simulink model "ForwardKinematic_YuMi"  (R2024a)
(part 12 of 23)

(9007199067919185*sin(q2L)*((5557241208790345*cos(q1L))/9007199254740992 - (6384186990310915*sin(q1L))/9007199254740992))/9007199254740992 - 347859890694807798813742879236295256254610072729/24519928653854221733733552434404946937899825954937634816)))/36893488147419103232000 + (81222263116692158804177042061221826384594597321566869716687*((9007199067919185*cos(q4L))/9007199254740992 - (234819211581865*sin(q4L))/1152921504606846976)*((432094733372955093709245836907320566011451687275*cos(q1L))/2993155353253689176481146537402947624255349848014848 - (499823478647255911063139966257565597426350154025*cos(q2L))/1461501637330902918203684832716283019655932542976 + (376125364442766701270516501597006072214248637825*sin(q1L))/2993155353253689176481146537402947624255349848014848 - (67682029681889335677290557259385*cos(q2L)*((6384186990310915*cos(q1L))/9007199254740992 + (5557241208790345*sin(q1L))/9007199254740992))/332306998946228968225951765070086144 + (9007199067919185*sin(q2L)*((5557241208790345*cos(q1L))/9007199254740992 - (6384186990310915*sin(q1L))/9007199254740992))/9007199254740992 - 347859890694807798813742879236295256254610072729/24519928653854221733733552434404946937899825954937634816))/306499108173177771671669405430061836723747824436720435200000 + (81*((234819211581865*cos(q4L))/1152921504606846976 + (9007199067919185*sin(q4L))/9007199254740992)*((432094733372955093709245836907320566011451687275*cos(q1L))/2993155353253689176481146537402947624255349848014848 - (499823478647255911063139966257565597426350154025*cos(q2L))/1461501637330902918203684832716283019655932542976 + (376125364442766701270516501597006072214248637825*sin(q1L))/2993155353253689176481146537402947624255349848014848 - (67682029681889335677290557259385*cos(q2L)*((6384186990310915*cos(q1L))/9007199254740992 + (5557241208790345*sin(q1L))/9007199254740992))/332306998946228968225951765070086144 + (9007199067919185*sin(q2L)*((5557241208790345*cos(q1L))/9007199254740992 - (6384186990310915*sin(q1L))/9007199254740992))/9007199254740992 - 347859890694807798813742879236295256254610072729/24519928653854221733733552434404946937899825954937634816))/2000,(48638874966763599*cos(q5L)*((783310804561232573774573497517025067305577458842146606386579375*cos(q2L))/55213970774324510299478046898216203619608871777363092441300193790394368 - (677168015718420743488926864722853474412798830140650728756148125*cos(q1L))/113078212145816597093331040047546785012958969400039613319782796882727665664 - (589454226189876320500100500762517606499114263738369612804244375*sin(q1L))/113078212145816597093331040047546785012958969400039613319782796882727665664 + (106069577339469832923929692356850887620017617375*cos(q2L)*((6384186990310915*cos(q1L))/9007199254740992 + (5557241208790345*sin(q1L))/9007199254740992))/12554203470773361527671578846415332832204710888928069025792 - (14115856197532180673579726082375*sin(q2L)*((5557241208790345*cos(q1L))/9007199254740992 - (6384186990310915*sin(q1L))/9007199254740992))/340282366920938463463374607431768211456 + (67682029681889335677290557259385*cos(q3L)*((55491554575214198102159220722265*cos(q2L))/162259276829213363391578010288128 + (7514214926474921*cos(q2L)*((6384186990310915*cos(q1L))/9007199254740992 + (5557241208790345*sin(q1L))/9007199254740992))/36893488147419103232 - sin(q2L)*((5557241208790345*cos(q1L))/9007199254740992 - (6384186990310915*sin(q1L))/9007199254740992)))/332306998946228968225951765070086144 + (234819211581865*cos(q3L)*((55491554575214198102159220722265*sin(q2L))/162259276829213363391578010288128 + cos(q2L)*((5557241208790345*cos(q1L))/9007199254740992 - (6384186990310915*sin(q1L))/9007199254740992) + (7514214926474921*sin(q2L)*((6384186990310915*cos(q1L))/9007199254740992 + (5557241208790345*sin(q1L))/9007199254740992))/36893488147419103232))/1152921504606846976 - (1764482024691522628700660907665*sin(q3L)*((55491554575214198102159220722265*cos(q2L))/162259276829213363391578010288128 + (7514214926474921*cos(q2L)*((6384186990310915*cos(q1L))/9007199254740992 + (5557241208790345*sin(q1L))/9007199254740992))/36893488147419103232 - sin(q2L)*((5557241208790345*cos(q1L))/9007199254740992 - (6384186990310915*sin(q1L))/9007199254740992)))/42535295865117307932921825928971026432 + (81129635049124235038645691064225*cos(q3L)*((57503643108550260546605243404275*cos(q1L))/81129638414606681695789005144064 + (50055177836018480443110068268825*sin(q1L))/81129638414606681695789005144064 - 46293577452674263141823442369649/664613997892457936451903530140172288))/81129638414606681695789005144064 + (9007199067919185*sin(q3L)*((55491554575214198102159220722265*sin(q2L))/162259276829213363391578010288128 + cos(q2L)*((5557241208790345*cos(q1L))/9007199254740992 - (6384186990310915*sin(q1L))/9007199254740992) + (7514214926474921*sin(q2L)*((6384186990310915*cos(q1L))/9007199254740992 + (5557241208790345*sin(q1L))/9007199254740992))/36893488147419103232))/9007199254740992 - (2115063383689692319117831580025*sin(q3L)*((57503643108550260546605243404275*cos(q1L))/81129638414606681695789005144064 + (50055177836018480443110068268825*sin(q1L))/81129638414606681695789005144064 - 46293577452674263141823442369649/664613997892457936451903530140172288))/10384593717069655257060992658440192 + 545157285512458543963749743061519108960107968042455893206992575/926336713898529563388567880069503262826159877325124512315660672063305037119488))/1801439850948198400 + (170695144106365826517608855445768431563113584343*sin(q5L)*((783310804561232573774573497517025067305577458842146606386579375*cos(q2L))/55213970774324510299478046898216203619608871777363092441300193790394368 - (677168015718420743488926864722853474412798830140650728756148125*cos(q1L))/113078212145816597093331040047546785012958969400039613319782796882727665664 - (589454226189876320500100500762517606499114263738369612804244375*sin(q1L))/113078212145816597093331040047546785012958969400039613319782796882727665664 + (106069577339469832923929692356850887620017617375*cos(q2L)*((6384186990310915*cos(q1L))/9007199254740992 + (5557241208790345*sin(q1L))/9007199254740992))/12554203470773361527671578846415332832204710888928069025792 - (14115856197532180673579726082375*sin(q2L)*((5557241208790345*cos(q1L))/9007199254740992 - (6384186990310915*sin(q1L))/9007199254740992))/340282366920938463463374607431768211456 + (67682029681889335677290557259385*cos(q3L)*((55491554575214198102159220722265*cos(q2L))/162259276829213363391578010288128 + (7514214926474921*cos(q2L)*((6384186990310915*cos(q1L))/9007199254740992 + (5557241208790345*sin(q1L))/9007199254740992))/36893488147419103232 - sin(q2L)*((5557241208790345*cos(q1L))/9007199254740992 - (6384186990310915*sin(q1L))/9007199254740992)))/332306998946228968225951765070086144 + (234819211581865*cos(q3L)*((55491554575214198102159220722265*sin(q2L))/162259276829213363391578010288128 + cos(q2L)*((5557241208790345*cos(q1L))/9007199254740992 - (6384186990310915*sin(q1L))/9007199254740992) + (7514214926474921*sin(q2L)*((6384186990310915*cos(q1L))/9007199254740992 + (5557241208790345*sin(q1L))/9007199254740992))/36893488147419103232))/1152921504606846976 - (1764482024691522628700660907665*sin(q3L)*((55491554575214198102159220722265*cos(q2L))/162259276829213363391578010288128 + (7514214926474921*cos(q2L)*((6384186990310915*cos(q1L))/9007199254740992 + (5557241208790345*sin(q1L))/9007199254740992))/36893488147419103232 - sin(q2L)*((5557241208790345*cos(q1L))/9007199254740992 - (6384186990310915*sin(q1L))/9007199254740992)))/42535295865117307932921825928971026432 + (81129635049124235038645691064225*cos(q3L)*((57503643108550260546605243404275*cos(q1L))/81129638414606681695789005144064 + (50055177836018480443110068268825*sin(q1L))/81129638414606681695789005144064 - 46293577452674263141823442369649/664613997892457936451903530140172288))/81129638414606681695789005144064 + (9007199067919185*sin(q3L)*((55491554575214198102159220722265*sin(q2L))/162259276829213363391578010288128 + cos(q2L)*((5557241208790345*cos(q1L))/9007199254740992 - (6384186990310915*sin(q1L))/9007199254740992) + (7514214926474921*sin(q2L)*((6384186990310915*cos(q1L))/9007199254740992 + (5557241208790345*sin(q1L))/9007199254740992))/36893488147419103232))/9007199254740992 - (2115063383689692319117831580025*sin(q3L)*((57503643108550260546605243404275*cos(q1L))/81129638414606681695789005144064 + (50055177836018480443110068268825*sin(q1L))/81129638414606681695789005144064 - 46293577452674263141823442369649/664613997892457936451903530140172288))/10384593717069655257060992658440192 + 545157285512458543963749743061519108960107968042455893206992575/926336713898529563388567880069503262826159877325124512315660672063305037119488))/119726214130147567059245861496117904970213993920593920 - (27*cos(q6L)*((9007199067919185*cos(q5L)*((783310804561232573774573497517025067305577458842146606386579375*cos(q2L))/55213970774324510299478046898216203619608871777363092441300193790394368 - (677168015718420743488926864722853474412798830140650728756148125*cos(q1L))/113078212145816597093331040047546785012958969400039613319782796882727665664 - (589454226189876320500100500762517606499114263738369612804244375*sin(q1L))/113078212145816597093331040047546785012958969400039613319782796882727665664 + (106069577339469832923929692356850887620017617375*cos(q2L)*((6384186990310915*cos(q1L))/9007199254740992 + (5557241208790345*sin(q1L))/9007199254740992))/12554203470773361527671578846415332832204710888928069025792 - (14115856197532180673579726082375*sin(q2L)*((5557241208790345*cos(q1L))/9007199254740992 - (6384186990310915*sin(q1L))/9007199254740992))/340282366920938463463374607431768211456 + (67682029681889335677290557259385*cos(q3L)*((55491554575214198102159220722265*cos(q2L))/162259276829213363391578010288128 + (7514214926474921*cos(q2L)*((6384186990310915*cos(q1L))/9007199254740992 + (5557241208790345*sin(q1L))/9007199254740992))/36893488147419103232 - sin(q2L)*((5557241208790345*cos(q1L))/9007199254740992 - (6384186990310915*sin(q1L))/9007199254740992)))/332306998946228968225951765070086144 + (234819211581865*cos(q3L)*((55491554575214198102159220722265*sin(q2L))/162259276829213363391578010288128 + cos(q2L)*((5557241208790345*cos(q1L))/9007199254740992 - (6384186990310915*sin(q1L))/9007199254740992) + (7514214926474921*sin(q2L)*((6384186990310915*cos(q1L))/9007199254740992 + (5557241208790345*sin(q1L))/9007199254740992))/36893488147419103232))/1152921504606846976 - (1764482024691522628700660907665*sin(q3L)*((55491554575214198102159220722265*cos(q2L))/162259276829213363391578010288128 + (7514214926474921*cos(q2L)*((6384186990310915*cos(q1L))/9007199254740992 + (5557241208790345*sin(q1L))/9007199254740992))/36893488147419103232 - sin(q2L)*((5557241208790345*cos(q1L))/9007199254740992 - (6384186990310915*sin(q1L))/9007199254740992)))/42535295865117307932921825928971026432 + (81129635049124235038645691064225*cos(q3L)*((57503643108550260546605243404275*cos(q1L))/81129638414606681695789005144064 + (50055177836018480443110068268825*sin(q1L))/81129638414606681695789005144064 - 46293577452674263141823442369649/664613997892457936451903530140172288))/81129638414606681695789005144064 + (9007199067919185*sin(q3L)*((55491554575214198102159220722265*sin(q2L))/162259276829213363391578010288128 + cos(q2L)*((5557241208790345*cos(q1L))/9007199254740992 - (6384186990310915*sin(q1L))/9007199254740992) + (7514214926474921*sin(q2L)*((6384186990310915*cos(q1L))/9007199254740992 + (5557241208790345*sin(q1L))/9007199254740992))/36893488147419103232))/9007199254740992 - (2115063383689692319117831580025*sin(q3L)*((57503643108550260546605243404275*cos(q1L))/81129638414606681695789005144064 + (50055177836018480443110068268825*sin(q1L))/81129638414606681695789005144064 - 46293577452674263141823442369649/664613997892457936451903530140172288))/10384593717069655257060992658440192 + 545157285512458543963749743061519108960107968042455893206992575/926336713898529563388567880069503262826159877325124512315660672063305037119488))/9007199254740992 + (7514214926474921*cos(q5L)*((7514214926474921*cos(q4L)*((7514214926474921*cos(q3L)*((55491554575214198102159220722265*cos(q2L))/162259276829213363391578010288128 + (7514214926474921*cos(q2L)*((6384186990310915*cos(q1L))/9007199254740992 + (5557241208790345*sin(q1L))/9007199254740992))/36893488147419103232 - sin(q2L)*((5557241208790345*cos(q1L))/9007199254740992 - (6384186990310915*sin(q1L))/9007199254740992)))/36893488147419103232 + (9007199067919185*cos(q3L)*((57503643108550260546605243404275*cos(q1L))/81129638414606681695789005144064 + (50055177836018480443110068268825*sin(q1L))/81129638414606681695789005144064 - 46293577452674263141823442369649/664613997892457936451903530140172288))/9007199254740992 + sin(q3L)*((55491554575214198102159220722265*sin(q2L))/162259276829213363391578010288128 + cos(q2L)*((5557241208790345*cos(q1L))/9007199254740992 - (6384186990310915*sin(q1L))/9007199254740992) + (7514214926474921*sin(q2L)*((6384186990310915*cos(q1L))/9007199254740992 + (5557241208790345*sin(q1L))/9007199254740992))/36893488147419103232)))/36893488147419103232 + ((4503599440548691*cos(q4L))/4503599627370496 - (7514214926474921*sin(q4L))/36893488147419103232)*((7514214926474921*sin(q3L)*((55491554575214198102159220722265*cos(q2L))/162259276829213363391578010288128 + (7514214926474921*cos(q2L)*((6384186990310915*cos(q1L))/9007199254740992 + (5557241208790345*sin(q1L))/9007199254740992))/36893488147419103232 - sin(q2L)*((5557241208790345*cos(q1L))/9007199254740992 - (6384186990310915*sin(q1L))/9007199254740992)))/36893488147419103232 - cos(q3L)*((55491554575214198102159220722265*sin(q2L))/162259276829213363391578010288128 + cos(q2L)*((5557241208790345*cos(q1L))/9007199254740992 - (6384186990310915*sin(q1L))/9007199254740992) + (7514214926474921*sin(q2L)*((6384186990310915*cos(q1L))/9007199254740992 + (5557241208790345*sin(q1L))/9007199254740992))/36893488147419103232) + (9007199067919185*sin(q3L)*((57503643108550260546605243404275*cos(q1L))/81129638414606681695789005144064 + (50055177836018480443110068268825*sin(q1L))/81129638414606681695789005144064 - 46293577452674263141823442369649/664613997892457936451903530140172288))/9007199254740992) + ((234819211581865*cos(q4L))/1152921504606846976 + (9007199067919185*sin(q4L))/9007199254740992)*((432094733372955093709245836907320566011451687275*cos(q1L))/2993155353253689176481146537402947624255349848014848 - (499823478647255911063139966257565597426350154025*cos(q2L))/1461501637330902918203684832716283019655932542976 + (376125364442766701270516501597006072214248637825*sin(q1L))/2993155353253689176481146537402947624255349848014848 - (67682029681889335677290557259385*cos(q2L)*((6384186990310915*cos(q1L))/9007199254740992 + (5557241208790345*sin(q1L))/9007199254740992))/332306998946228968225951765070086144 + (9007199067919185*sin(q2L)*((5557241208790345*cos(q1L))/9007199254740992 - (6384186990310915*sin(q1L))/9007199254740992))/9007199254740992 - 347859890694807798813742879236295256254610072729/24519928653854221733733552434404946937899825954937634816)))/36893488147419103232 + sin(q5L)*((7514214926474921*sin(q4L)*((7514214926474921*cos(q3L)*((55491554575214198102159220722265*cos(q2L))/162259276829213363391578010288128 + (7514214926474921*cos(q2L)*((6384186990310915*cos(q1L))/9007199254740992 + (5557241208790345*sin(q1L))/9007199254740992))/36893488147419103232 - sin(q2L)*((5557241208790345*cos(q1L))/9007199254740992 - (6384186990310915*sin(q1L))/9007199254740992)))/36893488147419103232 + (9007199067919185*cos(q3L)*((57503643108550260546605243404275*cos(q1L))/81129638414606681695789005144064 + (50055177836018480443110068268825*sin(q1L))/81129638414606681695789005144064 - 46293577452674263141823442369649/664613997892457936451903530140172288))/9007199254740992 + sin(q3L)*((55491554575214198102159220722265*sin(q2L))/162259276829213363391578010288128 + cos(q2L)*((5557241208790345*cos(q1L))/9007199254740992 - (6384186990310915*sin(q1L))/9007199254740992) + (7514214926474921*sin(q2L)*((6384186990310915*cos(q1L))/9007199254740992 + (5557241208790345*sin(q1L))/9007199254740992))/36893488147419103232)))/36893488147419103232 + ((7514214926474921*cos(q4L))/36893488147419103232 + (4503599440548691*sin(q4L))/4503599627370496)*((7514214926474921*sin(q3L)*((55491554575214198102159220722265*cos(q2L))/162259276829213363391578010288128 + (7514214926474921*cos(q2L)*((6384186990310915*cos(q1L))/9007199254740992 + (5557241208790345*sin(q1L))/9007199254740992))/36893488147419103232 - sin(q2L)*((5557241208790345*cos(q1L))/9007199254740992 - (6384186990310915*sin(q1L))/9007199254740992)))/36893488147419103232 - cos(q3L)*((55491554575214198102159220722265*sin(q2L))/162259276829213363391578010288128 + cos(q2L)*((5557241208790345*cos(q1L))/9007199254740992 - (6384186990310915*sin(q1L))/9007199254740992) + (7514214926474921*sin(q2L)*((6384186990310915*cos(q1L))/9007199254740992 + (5557241208790345*sin(q1L))/9007199254740992))/36893488147419103232) + (9007199067919185*sin(q3L)*((57503643108550260546605243404275*cos(q1L))/81129638414606681695789005144064 + (50055177836018480443110068268825*sin(q1L))/81129638414606681695789005144064 - 46293577452674263141823442369649/664613997892457936451903530140172288))/9007199254740992) - ((9007199067919185*cos(q4L))/9007199254740992 - (234819211581865*sin(q4L))/1152921504606846976)*((432094733372955093709245836907320566011451687275*cos(q1L))/2993155353253689176481146537402947624255349848014848 - (499823478647255911063139966257565597426350154025*cos(q2L))/1461501637330902918203684832716283019655932542976 + (376125364442766701270516501597006072214248637825*sin(q1L))/2993155353253689176481146537402947624255349848014848 - (67682029681889335677290557259385*cos(q2L)*((6384186990310915*cos(q1L))/9007199254740992 + (5557241208790345*sin(q1L))/9007199254740992))/332306998946228968225951765070086144 + (9007199067919185*sin(q2L)*((5557241208790345*cos(q1L))/9007199254740992 - (6384186990310915*sin(q1L))/9007199254740992))/9007199254740992 - 347859890694807798813742879236295256254610072729/24519928653854221733733552434404946937899825954937634816))))/1000 + (324259171862923063*sin(q6L)*((9007199067919185*cos(q5L)*((783310804561232573774573497517025067305577458842146606386579375*cos(q2L))/55213970774324510299478046898216203619608871777363092441300193790394368 - (677168015718420743488926864722853474412798830140650728756148125*cos(q1L))/113078212145816597093331040047546785012958969400039613319782796882727665664 - (589454226189876320500100500762517606499114263738369612804244375*sin(q1L))/113078212145816597093331040047546785012958969400039613319782796882727665664 + (106069577339469832923929692356850887620017617375*cos(q2L)*((6384186990310915*cos(q1L))/9007199254740992 + (5557241208790345*sin(q1L))/9007199254740992))/12554203470773361527671578846415332832204710888928069025792 - (14115856197532180673579726082375*sin(q2L)*((5557241208790345*cos(q1L))/9007199254740992 - (6384186990310915*sin(q1L))/9007199254740992))/340282366920938463463374607431768211456 + (67682029681889335677290557259385*cos(q3L)*((55491554575214198102159220722265*cos(q2L))/162259276829213363391578010288128 + (7514214926474921*cos(q2L)*((6384186990310915*cos(q1L))/9007199254740992 + (5557241208790345*sin(q1L))/9007199254740992))/36893488147419103232 - sin(q2L)*((5557241208790345*cos(q1L))/9007199254740992 - (6384186990310915*sin(q1L))/9007199254740992)))/332306998946228968225951765070086144 + (234819211581865*cos(q3L)*((55491554575214198102159220722265*sin(q2L))/162259276829213363391578010288128 + cos(q2L)*((5557241208790345*cos(q1L))/9007199254740992 - (6384186990310915*sin(q1L))/9007199254740992) + (7514214926474921*sin(q2L)*((6384186990310915*cos(q1L))/9007199254740992 + (5557241208790345*sin(q1L))/9007199254740992))/36893488147419103232))/1152921504606846976 - (1764482024691522628700660907665*sin(q3L)*((55491554575214198102159220722265*cos(q2L))/162259276829213363391578010288128 + (7514214926474921*cos(q2L)*((6384186990310915*cos(q1L))/9007199254740992 + (5557241208790345*sin(q1L))/9007199254740992))/36893488147419103232 - sin(q2L)*((5557241208790345*cos(q1L))/9007199254740992 - (6384186990310915*sin(q1L))/9007199254740992)))/42535295865117307932921825928971026432 + (81129635049124235038645691064225*cos(q3L)*((57503643108550260546605243404275*cos(q1L))/81129638414606681695789005144064 + (50055177836018480443110068268825*sin(q1L))/81129638414606681695789005144064 - 46293577452674263141823442369649/664613997892457936451903530140172288))/81129638414606681695789005144064 + (9007199067919185*sin(q3L)*((55491554575214198102159220722265*sin(q2L))/162259276829213363391578010288128 + cos(q2L)*((5557241208790345*cos(q1L))/9007199254740992 - (6384186990310915*sin(q1L))/9007199254740992) + (7514214926474921*sin(q2L)*((6384186990310915*cos(q1L))/9007199254740992 + (5557241208790345*sin(q1L))/9007199254740992))/36893488147419103232))/9007199254740992 - (2115063383689692319117831580025*sin(q3L)*((57503643108550260546605243404275*cos(q1L))/81129638414606681695789005144064 + (50055177836018480443110068268825*sin(q1L))/81129638414606681695789005144064 - 46293577452674263141823442369649/664613997892457936451903530140172288))/10384593717069655257060992658440192 + 545157285512458543963749743061519108960107968042455893206992575/926336713898529563388567880069503262826159877325124512315660672063305037119488))/9007199254740992 + (7514214926474921*cos(q5L)*((7514214926474921*cos(q4L)*((7514214926474921*cos(q3L)*((55491554575214198102159220722265*cos(q2L))/162259276829213363391578010288128 + (7514214926474921*cos(q2L)*((6384186990310915*cos(q1L))/9007199254740992 + (5557241208790345*sin(q1L))/9007199254740992))/36893488147419103232 - sin(q2L)*((5557241208790345*cos(q1L))/9007199254740992 - (6384186990310915*sin(q1L))/9007199254740992)))/36893488147419103232 + (9007199067919185*cos(q3L)*((57503643108550260546605243404275*cos(q1L))/81129638414606681695789005144064 + (50055177836018480443110068268825*sin(q1L))/81129638414606681695789005144064 - 46293577452674263141823442369649/664613997892457936451903530140172288))/9007199254740992 + sin(q3L)*((55491554575214198102159220722265*sin(q2L))/162259276829213363391578010288128 + cos(q2L)*((5557241208790345*cos(q1L))/9007199254740992 - (6384186990310915*sin(q1L))/9007199254740992) + (7514214926474921*sin(q2L)*((6384186990310915*cos(q1L))/9007199254740992 + (5557241208790345*sin(q1L))/9007199254740992))/36893488147419103232)))/36893488147419103232 + ((4503599440548691*cos(q4L))/4503599627370496 - (7514214926474921*sin(q4L))/36893488147419103232)*((7514214926474921*sin(q3L)*((55491554575214198102159220722265*cos(q2L))/162259276829213363391578010288128 + (7514214926474921*cos(q2L)*((6384186990310915*cos(q1L))/9007199254740992 + (5557241208790345*sin(q1L))/9007199254740992))/36893488147419103232 - sin(q2L)*((5557241208790345*cos(q1L))/9007199254740992 - (6384186990310915*sin(q1L))/9007199254740992)))/36893488147419103232 - cos(q3L)*((55491554575214198102159220722265*sin(q2L))/162259276829213363391578010288128 + cos(q2L)*((5557241208790345*cos(q1L))/9007199254740992 - (6384186990310915*sin(q1L))/9007199254740992) + (7514214926474921*sin(q2L)*((6384186990310915*cos(q1L))/9007199254740992 + (5557241208790345*sin(q1L))/9007199254740992))/36893488147419103232) + (9007199067919185*sin(q3L)*((57503643108550260546605243404275*cos(q1L))/81129638414606681695789005144064 + (50055177836018480443110068268825*sin(q1L))/81129638414606681695789005144064 - 46293577452674263141823442369649/664613997892457936451903530140172288))/9007199254740992) + ((234819211581865*cos(q4L))/1152921504606846976 + (9007199067919185*sin(q4L))/9007199254740992)*((432094733372955093709245836907320566011451687275*cos(q1L))/2993155353253689176481146537402947624255349848014848 - (499823478647255911063139966257565597426350154025*cos(q2L))/1461501637330902918203684832716283019655932542976 + (376125364442766701270516501597006072214248637825*sin(q1L))/2993155353253689176481146537402947624255349848014848 - (67682029681889335677290557259385*cos(q2L)*((6384186990310915*cos(q1L))/9007199254740992 + (5557241208790345*sin(q1L))/9007199254740992))/332306998946228968225951765070086144 + (9007199067919185*sin(q2L)*((5557241208790345*cos(q1L))/9007199254740992 - (6384186990310915*sin(q1L))/9007199254740992))/9007199254740992 - 347859890694807798813742879236295256254610072729/24519928653854221733733552434404946937899825954937634816)))/36893488147419103232 + sin(q5L)*((7514214926474921*sin(q4L)*((7514214926474921*cos(q3L)*((55491554575214198102159220722265*cos(q2L))/162259276829213363391578010288128 + (7514214926474921*cos(q2L)*((6384186990310915*cos(q1L))/9007199254740992 + (5557241208790345*sin(q1L))/9007199254740992))/36893488147419103232 - sin(q2L)*((5557241208790345*cos(q1L))/9007199254740992 - (6384186990310915*sin(q1L))/9007199254740992)))/36893488147419103232 + (9007199067919185*cos(q3L)*((57503643108550260546605243404275*cos(q1L))/81129638414606681695789005144064 + (50055177836018480443110068268825*sin(q1L))/81129638414606681695789005144064 - 46293577452674263141823442369649/664613997892457936451903530140172288))/9007199254740992 + sin(q3L)*((55491554575214198102159220722265*sin(q2L))/162259276829213363391578010288128 + cos(q2L)*((5557241208790345*cos(q1L))/9007199254740992 - (6384186990310915*sin(q1L))/9007199254740992) + (7514214926474921*sin(q2L)*((6384186990310915*cos(q1L))/9007199254740992 + (5557241208790345*sin(q1L))/9007199254740992))/36893488147419103232)))/36893488147419103232 + ((7514214926474921*cos(q4L))/36893488147419103232 + (4503599440548691*sin(q4L))/4503599627370496)*((7514214926474921*sin(q3L)*((55491554575214198102159220722265*cos(q2L))/162259276829213363391578010288128 + (7514214926474921*cos(q2L)*((6384186990310915*cos(q1L))/9007199254740992 + (5557241208790345*sin(q1L))/9007199254740992))/36893488147419103232 - sin(q2L)*((5557241208790345*cos(q1L))/9007199254740992 - (6384186990310915*sin(q1L))/9007199254740992)))/36893488147419103232 - cos(q3L)*((55491554575214198102159220722265*sin(q2L))/162259276829213363391578010288128 + cos(q2L)*((5557241208790345*cos(q1L))/9007199254740992 - (6384186990310915*sin(q1L))/9007199254740992) + (7514214926474921*sin(q2L)*((6384186990310915*cos(q1L))/9007199254740992 + (5557241208790345*sin(q1L))/9007199254740992))/36893488147419103232) + (9007199067919185*sin(q3L)*((57503643108550260546605243404275*cos(q1L))/81129638414606681695789005144064 + (50055177836018480443110068268825*sin(q1L))/81129638414606681695789005144064 - 46293577452674263141823442369649/664613997892457936451903530140172288))/9007199254740992) - ((9007199067919185*cos(q4L))/9007199254740992 - (234819211581865*sin(q4L))/1152921504606846976)*((432094733372955093709245836907320566011451687275*cos(q1L))/2993155353253689176481146537402947624255349848014848 - (499823478647255911063139966257565597426350154025*cos(q2L))/1461501637330902918203684832716283019655932542976 + (376125364442766701270516501597006072214248637825*sin(q1L))/2993155353253689176481146537402947624255349848014848 - (67682029681889335677290557259385*cos(q2L)*((6384186990310915*cos(q1L))/9007199254740992 + (5557241208790345*sin(q1L))/9007199254740992))/332306998946228968225951765070086144 + (9007199067919185*sin(q2L)*((5557241208790345*cos(q1L))/9007199254740992 - (6384186990310915*sin(q1L))/9007199254740992))/9007199254740992 - 347859890694807798813742879236295256254610072729/24519928653854221733733552434404946937899825954937634816))))/9007199254740992000 - (2436553109258773196144549622003023*cos(q6L)*((9007199067919185*sin(q5L)*((783310804561232573774573497517025067305577458842146606386579375*cos(q2L))/55213970774324510299478046898216203619608871777363092441300193790394368 - (677168015718420743488926864722853474412798830140650728756148125*cos(q1L))/113078212145816597093331040047546785012958969400039613319782796882727665664 - (589454226189876320500100500762517606499114263738369612804244375*sin(q1L))/113078212145816597093331040047546785012958969400039613319782796882727665664 + (106069577339469832923929692356850887620017617375*cos(q2L)*((6384186990310915*cos(q1L))/9007199254740992 + (5557241208790345*sin(q1L))/9007199254740992))/12554203470773361527671578846415332832204710888928069025792 - (14115856197532180673579726082375*sin(q2L)*((5557241208790345*cos(q1L))/9007199254740992 - (6384186990310915*sin(q1L))/9007199254740992))/340282366920938463463374607431768211456 + (67682029681889335677290557259385*cos(q3L)*((55491554575214198102159220722265*cos(q2L))/162259276829213363391578010288128 + (7514214926474921*cos(q2L)*((6384186990310915*cos(q1L))/9007199254740992 + (5557241208790345*sin(q1L))/9007199254740992))/36893488147419103232 - sin(q2L)*((5557241208790345*cos(q1L))/9007199254740992 - (6384186990310915*sin(q1L))/9007199254740992)))/332306998946228968225951765070086144 + (234819211581865*cos(q3L)*((55491554575214198102159220722265*sin(q2L))/162259276829213363391578010288128 + cos(q2L)*((5557241208790345*cos(q1L))/9007199254740992 - (6384186990310915*sin(q1L))/9007199254740992) + (7514214926474921*sin(q2L)*((6384186990310915*cos(q1L))/9007199254740992 + (5557241208790345*sin(q1L))/9007199254740992))/36893488147419103232))/1152921504606846976 - (1764482024691522628700660907665*sin(q3L)*((55491554575214198102159220722265*cos(q2L))/162259276829213363391578010288128 + (7514214926474921*cos(q2L)*((6384186990310915*cos(q1L))/9007199254740992 + (5557241208790345*sin(q1L))/9007199254740992))/36893488147419103232 - sin(q2L)*((5557241208790345*cos(q1L))/9007199254740992 - (6384186990310915*sin(q1L))/9007199254740992)))/42535295865117307932921825928971026432 + (81129635049124235038645691064225*cos(q3L)*((57503643108550260546605243404275*cos(q1L))/81129638414606681695789005144064 + (50055177836018480443110068268825*sin(q1L))/81129638414606681695789005144064 - 46293577452674263141823442369649/664613997892457936451903530140172288))/81129638414606681695789005144064 + (9007199067919185*sin(q3L)*((55491554575214198102159220722265*sin(q2L))/162259276829213363391578010288128 + cos(q2L)*((5557241208790345*cos(q1L))/9007199254740992 - (6384186990310915*sin(q1L))/9007199254740992) + (7514214926474921*sin(q2L)*((6384186990310915*cos(q1L))/9007199254740992 + (5557241208790345*sin(q1L))/9007199254740992))/36893488147419103232))/9007199254740992 - (2115063383689692319117831580025*sin(q3L)*((57503643108550260546605243404275*cos(q1L))/81129638414606681695789005144064 + (50055177836018480443110068268825*sin(q1L))/81129638414606681695789005144064 - 46293577452674263141823442369649/664613997892457936451903530140172288))/10384593717069655257060992658440192 + 545157285512458543963749743061519108960107968042455893206992575/926336713898529563388567880069503262826159877325124512315660672063305037119488))/9007199254740992 + (7514214926474921*sin(q5L)*((7514214926474921*cos(q4L)*((7514214926474921*cos(q3L)*((55491554575214198102159220722265*cos(q2L))/162259276829213363391578010288128 + (7514214926474921*cos(q2L)*((6384186990310915*cos(q1L))/9007199254740992 + (5557241208790345*sin(q1L))/9007199254740992))/36893488147419103232 - sin(q2L)*((5557241208790345*cos(q1L))/9007199254740992 - (6384186990310915*sin(q1L))/9007199254740992)))/36893488147419103232 + (9007199067919185*cos(q3L)*((57503643108550260546605243404275*cos(q1L))/81129638414606681695789005144064 + (50055177836018480443110068268825*sin(q1L))/81129638414606681695789005144064 - 46293577452674263141823442369649/664613997892457936451903530140172288))/9007199254740992 + sin(q3L)*((55491554575214198102159220722265*sin(q2L))/162259276829213363391578010288128 + cos(q2L)*((5557241208790345*cos(q1L))/9007199254740992 - (6384186990310915*sin(q1L))/9007199254740992) + (7514214926474921*sin(q2L)*((6384186990310915*cos(q1L))/9007199254740992 + (5557241208790345*sin(q1L))/9007199254740992))/36893488147419103232)))/36893488147419103232 + ((4503599440548691*cos(q4L))/4503599627370496 - (7514214926474921*sin(q4L))/36893488147419103232)*((7514214926474921*sin(q3L)*((55491554575214198102159220722265*cos(q2L))/162259276829213363391578010288128 + (7514214926474921*cos(q2L)*((6384186990310915*cos(q1L))/9007199254740992 + (5557241208790345*sin(q1L))/9007199254740992))/36893488147419103232 - sin(q2L)*((5557241208790345*cos(q1L))/9007199254740992 - (6384186990310915*sin(q1L))/9007199254740992)))/36893488147419103232 - cos(q3L)*((55491554575214198102159220722265*sin(q2L))/162259276829213363391578010288128 + cos(q2L)*((5557241208790345*cos(q1L))/9007199254740992 - (6384186990310915*sin(q1L))/9007199254740992) + (7514214926474921*sin(q2L)*((6384186990310915*cos(q1L))/9007199254740992 + (5557241208790345*sin(q1L))/9007199254740992))/36893488147419103232) + (9007199067919185*sin(q3L)*((57503643108550260546605243404275*cos(q1L))/81129638414606681695789005144064 + (50055177836018480443110068268825*sin(q1L))/81129638414606681695789005144064 - 46293577452674263141823442369649/664613997892457936451903530140172288))/9007199254740992) + ((234819211581865*cos(q4L))/1152921504606846976 + (9007199067919185*sin(q4L))/9007199254740992)*((432094733372955093709245836907320566011451687275*cos(q1L))/2993155353253689176481146537402947624255349848014848 - (499823478647255911063139966257565597426350154025*cos(q2L))/1461501637330902918203684832716283019655932542976 + (376125364442766701270516501597006072214248637825*sin(q1L))/2993155353253689176481146537402947624255349848014848 - (67682029681889335677290557259385*cos(q2L)*((6384186990310915*cos(q1L))/9007199254740992 + (5557241208790345*sin(q1L))/9007199254740992))/332306998946228968225951765070086144 + (9007199067919185*sin(q2L)*((5557241208790345*cos(q1L))/9007199254740992 - (6384186990310915*sin(q1L))/9007199254740992))/9007199254740992 - 347859890694807798813742879236295256254610072729/24519928653854221733733552434404946937899825954937634816)))/36893488147419103232 - cos(q5L)*((7514214926474921*sin(q4L)*((7514214926474921*cos(q3L)*((55491554575214198102159220722265*cos(q2L))/162259276829213363391578010288128 + (7514214926474921*cos(q2L)*((6384186990310915*cos(q1L))/9007199254740992 + (5557241208790345*sin(q1L))/9007199254740992))/36893488147419103232 - sin(q2L)*((5557241208790345*cos(q1L))/9007199254740992 - (6384186990310915*sin(q1L))/9007199254740992)))/36893488147419103232 + (9007199067919185*cos(q3L)*((57503643108550260546605243404275*cos(q1L))/81129638414606681695789005144064 + (50055177836018480443110068268825*sin(q1L))/81129638414606681695789005144064 - 46293577452674263141823442369649/664613997892457936451903530140172288))/9007199254740992 + sin(q3L)*((55491554575214198102159220722265*sin(q2L))/162259276829213363391578010288128 + cos(q2L)*((5557241208790345*cos(q1L))/9007199254740992 - (6384186990310915*sin(q1L))/9007199254740992) + (7514214926474921*sin(q2L)*((6384186990310915*cos(q1L))/9007199254740992 + (5557241208790345*sin(q1L))/9007199254740992))/36893488147419103232)))/36893488147419103232 + ((7514214926474921*cos(q4L))/36893488147419103232 + (4503599440548691*sin(q4L))/4503599627370496)*((7514214926474921*sin(q3L)*((55491554575214198102159220722265*cos(q2L))/162259276829213363391578010288128 + (7514214926474921*cos(q2L)*((6384186990310915*cos(q1L))/9007199254740992 + (5557241208790345*sin(q1L))/9007199254740992))/36893488147419103232 - sin(q2L)*((5557241208790345*cos(q1L))/9007199254740992 - (6384186990310915*sin(q1L))/9007199254740992)))/36893488147419103232 - cos(q3L)*((55491554575214198102159220722265*sin(q2L))/162259276829213363391578010288128 + cos(q2L)*((5557241208790345*cos(q1L))/9007199254740992 - (6384186990310915*sin(q1L))/9007199254740992) + (7514214926474921*sin(q2L)*((6384186990310915*cos(q1L))/9007199254740992 + (5557241208790345*sin(q1L))/9007199254740992))/36893488147419103232) + (9007199067919185*sin(q3L)*((57503643108550260546605243404275*cos(q1L))/81129638414606681695789005144064 + (50055177836018480443110068268825*sin(q1L))/81129638414606681695789005144064 - 46293577452674263141823442369649/664613997892457936451903530140172288))/9007199254740992) - ((9007199067919185*cos(q4L))/9007199254740992 - (234819211581865*sin(q4L))/1152921504606846976)*((432094733372955093709245836907320566011451687275*cos(q1L))/2993155353253689176481146537402947624255349848014848 - (499823478647255911063139966257565597426350154025*cos(q2L))/1461501637330902918203684832716283019655932542976 + (376125364442766701270516501597006072214248637825*sin(q1L))/2993155353253689176481146537402947624255349848014848 - (67682029681889335677290557259385*cos(q2L)*((6384186990310915*cos(q1L))/9007199254740992 + (5557241208790345*sin(q1L))/9007199254740992))/332306998946228968225951765070086144 + (9007199067919185*sin(q2L)*((5557241208790345*cos(q1L))/9007199254740992 - (6384186990310915*sin(q1L))/9007199254740992))/9007199254740992 - 347859890694807798813742879236295256254610072729/24519928653854221733733552434404946937899825954937634816))))/332306998946228968225951765070086144000 - (202883803014822867*sin(q6L)*((9007199067919185*sin(q5L)*((783310804561232573774573497517025067305577458842146606386579375*cos(q2L))/55213970774324510299478046898216203619608871777363092441300193790394368 - (677168015718420743488926864722853474412798830140650728756148125*cos(q1L))/113078212145816597093331040047546785012958969400039613319782796882727665664 - (589454226189876320500100500762517606499114263738369612804244375*sin(q1L))/113078212145816597093331040047546785012958969400039613319782796882727665664 + (106069577339469832923929692356850887620017617375*cos(q2L)*((6384186990310915*cos(q1L))/9007199254740992 + (5557241208790345*sin(q1L))/9007199254740992))/12554203470773361527671578846415332832204710888928069025792 - (14115856197532180673579726082375*sin(q2L)*((5557241208790345*cos(q1L))/9007199254740992 - (6384186990310915*sin(q1L))/9007199254740992))/340282366920938463463374607431768211456 + (67682029681889335677290557259385*cos(q3L)*((55491554575214198102159220722265*cos(q2L))/162259276829213363391578010288128 + (7514214926474921*cos(q2L)*((6384186990310915*cos(q1L))/9007199254740992 + (5557241208790345*sin(q1L))/9007199254740992))/36893488147419103232 - sin(q2L)*((5557241208790345*cos(q1L))/9007199254740992 - (6384186990310915*sin(q1L))/9007199254740992)))/332306998946228968225951765070086144 + (234819211581865*cos(q3L)*((55491554575214198102159220722265*sin(q2L))/162259276829213363391578010288128 + cos(q2L)*((5557241208790345*cos(q1L))/9007199254740992 - (6384186990310915*sin(q1L))/9007199254740992) + (7514214926474921*sin(q2L)*((6384186990310915*cos(q1L))/9007199254740992 + (5557241208790345*sin(q1L))/9007199254740992))/36893488147419103232))/1152921504606846976 - (1764482024691522628700660907665*sin(q3L)*((55491554575214198102159220722265*cos(q2L))/162259276829213363391578010288128 + (7514214926474921*cos(q2L)*((6384186990310915*cos(q1L))/9007199254740992 + (5557241208790345*sin(q1L))/9007199254740992))/36893488147419103232 - sin(q2L)*((5557241208790345*cos(q1L))/9007199254740992 - (6384186990310915*sin(q1L))/9007199254740992)))/42535295865117307932921825928971026432 + (81129635049124235038645691064225*cos(q3L)*((57503643108550260546605243404275*cos(q1L))/81129638414606681695789005144064 + (50055177836018480443110068268825*sin(q1L))/81129638414606681695789005144064 - 46293577452674263141823442369649/664613997892457936451903530140172288))/81129638414606681695789005144064 + (9007199067919185*sin(q3L)*((55491554575214198102159220722265*sin(q2L))/162259276829213363391578010288128 + cos(q2L)*((5557241208790345*cos(q1L))/9007199254740992 - (6384186990310915*sin(q1L))/9007199254740992) + (7514214926474921*sin(q2L)*((6384186990310915*cos(q1L))/9007199254740992 + (5557241208790345*sin(q1L))/9007199254740992))/36893488147419103232))/9007199254740992 - (2115063383689692319117831580025*sin(q3L)*((57503643108550260546605243404275*cos(q1L))/81129638414606681695789005144064 + (50055177836018480443110068268825*sin(q1L))/81129638414606681695789005144064 - 46293577452674263141823442369649/664613997892457936451903530140172288))/10384593717069655257060992658440192 + 545157285512458543963749743061519108960107968042455893206992575/926336713898529563388567880069503262826159877325124512315660672063305037119488))/9007199254740992 + (7514214926474921*sin(q5L)*((7514214926474921*cos(q4L)*((7514214926474921*cos(q3L)*((55491554575214198102159220722265*cos(q2L))/162259276829213363391578010288128 + (7514214926474921*cos(q2L)*((6384186990310915*cos(q1L))/9007199254740992 + (5557241208790345*sin(q1L))/9007199254740992))/36893488147419103232 - sin(q2L)*((5557241208790345*cos(q1L))/9007199254740992 - (6384186990310915*sin(q1L))/9007199254740992)))/36893488147419103232 + (9007199067919185*cos(q3L)*((57503643108550260546605243404275*cos(q1L))/81129638414606681695789005144064 + (50055177836018480443110068268825*sin(q1L))/81129638414606681695789005144064 - 46293577452674263141823442369649/664613997892457936451903530140172288))/9007199254740992 + sin(q3L)*((55491554575214198102159220722265*sin(q2L))/162259276829213363391578010288128 + cos(q2L)*((5557241208790345*cos(q1L))/9007199254740992 - (6384186990310915*sin(q1L))/9007199254740992) + (7514214926474921*sin(q2L)*((6384186990310915*cos(q1L))/9007199254740992 + (5557241208790345*sin(q1L))/9007199254740992))/36893488147419103232)))/36893488147419103232 + ((4503599440548691*cos(q4L))/4503599627370496 - (7514214926474921*sin(q4L))/36893488147419103232)*((7514214926474921*sin(q3L)*((55491554575214198102159220722265*cos(q2L))/162259276829213363391578010288128 + (7514214926474921*cos(q2L)*((6384186990310915*cos(q1L))/9007199254740992 + (5557241208790345*sin(q1L))/9007199254740992))/36893488147419103232 - sin(q2L)*((5557241208790345*cos(q1L))/9007199254740992 - (6384186990310915*sin(q1L))/9007199254740992)))/36893488147419103232 - cos(q3L)*((55491554575214198102159220722265*sin(q2L))/162259276829213363391578010288128 + cos(q2L)*((5557241208790345*cos(q1L))/9007199254740992 - (6384186990310915*sin(q1L))/9007199254740992) + (7514214926474921*sin(q2L)*((6384186990310915*cos(q1L))/9007199254740992 + (5557241208790345*sin(q1L))/9007199254740992))/36893488147419103232) + (9007199067919185*sin(q3L)*((57503643108550260546605243404275*cos(q1L))/81129638414606681695789005144064 + (50055177836018480443110068268825*sin(q1L))/81129638414606681695789005144064 - 46293577452674263141823442369649/664613997892457936451903530140172288))/9007199254740992) + ((234819211581865*cos(q4L))/1152921504606846976 + (9007199067919185*sin(q4L))/9007199254740992)*((432094733372955093709245836907320566011451687275*cos(q1L))/2993155353253689176481146537402947624255349848014848 - (499823478647255911063139966257565597426350154025*cos(q2L))/1461501637330902918203684832716283019655932542976 + (376125364442766701270516501597006072214248637825*sin(q1L))/2993155353253689176481146537402947624255349848014848 - (67682029681889335677290557259385*cos(q2L)*((6384186990310915*cos(q1L))/9007199254740992 + (5557241208790345*sin(q1L))/9007199254740992))/332306998946228968225951765070086144 + (9007199067919185*sin(q2L)*((5557241208790345*cos(q1L))/9007199254740992 - (6384186990310915*sin(q1L))/9007199254740992))/9007199254740992 - 347859890694807798813742879236295256254610072729/24519928653854221733733552434404946937899825954937634816)))/36893488147419103232 - cos(q5L)*((7514214926474921*sin(q4L)*((7514214926474921*cos(q3L)*((55491554575214198102159220722265*cos(q2L))/162259276829213363391578010288128 + (7514214926474921*cos(q2L)*((6384186990310915*cos(q1L))/9007199254740992 + (5557241208790345*sin(q1L))/9007199254740992))/36893488147419103232 - sin(q2L)*((5557241208790345*cos(q1L))/9007199254740992 - (6384186990310915*sin(q1L))/9007199254740992)))/36893488147419103232 + (9007199067919185*cos(q3L)*((57503643108550260546605243404275*cos(q1L))/81129638414606681695789005144064 + (50055177836018480443110068268825*sin(q1L))/81129638414606681695789005144064 - 46293577452674263141823442369649/664613997892457936451903530140172288))/9007199254740992 + sin(q3L)*((55491554575214198102159220722265*sin(q2L))/162259276829213363391578010288128 + cos(q2L)*((5557241208790345*cos(q1L))/9007199254740992 - (6384186990310915*sin(q1L))/9007199254740992) + (7514214926474921*sin(q2L)*((6384186990310915*cos(q1L))/9007199254740992 + (5557241208790345*sin(q1L))/9007199254740992))/36893488147419103232)))/36893488147419103232 + ((7514214926474921*cos(q4L))/36893488147419103232 + (4503599440548691*sin(q4L))/4503599627370496)*((7514214926474921*sin(q3L)*((55491554575214198102159220722265*cos(q2L))/162259276829213363391578010288128 + (7514214926474921*cos(q2L)*((6384186990310915*cos(q1L))/9007199254740992 + (5557241208790345*sin(q1L))/9007199254740992))/36893488147419103232 - sin(q2L)*((5557241208790345*cos(q1L))/9007199254740992 - (6384186990310915*sin(q1L))/9007199254740992)))/36893488147419103232 - cos(q3L)*((55491554575214198102159220722265*sin(q2L))/162259276829213363391578010288128 + cos(q2L)*((5557241208790345*cos(q1L))/9007199254740992 - (6384186990310915*sin(q1L))/9007199254740992) + (7514214926474921*sin(q2L)*((6384186990310915*cos(q1L))/9007199254740992 + (5557241208790345*sin(q1L))/9007199254740992))/36893488147419103232) + (9007199067919185*sin(q3L)*((57503643108550260546605243404275*cos(q1L))/81129638414606681695789005144064 + (50055177836018480443110068268825*sin(q1L))/81129638414606681695789005144064 - 46293577452674263141823442369649/664613997892457936451903530140172288))/9007199254740992) - ((9007199067919185*cos(q4L))/9007199254740992 - (234819211581865*sin(q4L))/1152921504606846976)*((432094733372955093709245836907320566011451687275*cos(q1L))/2993155353253689176481146537402947624255349848014848 - (499823478647255911063139966257565597426350154025*cos(q2L))/1461501637330902918203684832716283019655932542976 + (376125364442766701270516501597006072214248637825*sin(q1L))/2993155353253689176481146537402947624255349848014848 - (67682029681889335677290557259385*cos(q2L)*((6384186990310915*cos(q1L))/9007199254740992 + (5557241208790345*sin(q1L))/9007199254740992))/332306998946228968225951765070086144 + (9007199067919185*sin(q2L)*((5557241208790345*cos(q1L))/9007199254740992 - (6384186990310915*sin(q1L))/9007199254740992))/9007199254740992 - 347859890694807798813742879236295256254610072729/24519928653854221733733552434404946937899825954937634816))))/36893488147419103232000 + (202883803014822867*cos(q5L)*((7514214926474921*cos(q4L)*((7514214926474921*cos(q3L)*((55491554575214198102159220722265*cos(q2L))/162259276829213363391578010288128 + (7514214926474921*cos(q2L)*((6384186990310915*cos(q1L))/9007199254740992 + (5557241208790345*sin(q1L))/9007199254740992))/36893488147419103232 - sin(q2L)*((5557241208790345*cos(q1L))/9007199254740992 - (6384186990310915*sin(q1L))/9007199254740992)))/36893488147419103232 + (9007199067919185*cos(q3L)*((57503643108550260546605243404275*cos(q1L))/81129638414606681695789005144064 + (50055177836018480443110068268825*sin(q1L))/81129638414606681695789005144064 - 46293577452674263141823442369649/664613997892457936451903530140172288))/9007199254740992 + sin(q3L)*((55491554575214198102159220722265*sin(q2L))/162259276829213363391578010288128 + cos(q2L)*((5557241208790345*cos(q1L))/9007199254740992 - (6384186990310915*sin(q1L))/9007199254740992) + (7514214926474921*sin(q2L)*((6384186990310915*cos(q1L))/9007199254740992 + (5557241208790345*sin(q1L))/9007199254740992))/36893488147419103232)))/36893488147419103232 + ((4503599440548691*cos(q4L))/4503599627370496 - (7514214926474921*sin(q4L))/36893488147419103232)*((7514214926474921*sin(q3L)*((55491554575214198102159220722265*cos(q2L))/162259276829213363391578010288128 + (7514214926474921*cos(q2L)*((6384186990310915*cos(q1L))/9007199254740992 + (5557241208790345*sin(q1L))/9007199254740992))/36893488147419103232 - sin(q2L)*((5557241208790345*cos(q1L))/9007199254740992 - (6384186990310915*sin(q1L))/9007199254740992)))/36893488147419103232 - cos(q3L)*((55491554575214198102159220722265*sin(q2L))/162259276829213363391578010288128 + cos(q2L)*((5557241208790345*cos(q1L))/9007199254740992 - (6384186990310915*sin(q1L))/9007199254740992) + (7514214926474921*sin(q2L)*((6384186990310915*cos(q1L))/9007199254740992 + (5557241208790345*sin(q1L))/9007199254740992))/36893488147419103232) + (9007199067919185*sin(q3L)*((57503643108550260546605243404275*cos(q1L))/81129638414606681695789005144064 + (50055177836018480443110068268825*sin(q1L))/81129638414606681695789005144064 - 46293577452674263141823442369649/664613997892457936451903530140172288))/9007199254740992) + ((234819211581865*cos(q4L))/1152921504606846976 + (9007199067919185*sin(q4L))/9007199254740992)*((432094733372955093709245836907320566011451687275*cos(q1L))/2993155353253689176481146537402947624255349848014848 - (499823478647255911063139966257565597426350154025*cos(q2L))/1461501637330902918203684832716283019655932542976 + (376125364442766701270516501597006072214248637825*sin(q1L))/2993155353253689176481146537402947624255349848014848 - (67682029681889335677290557259385*cos(q2L)*((6384186990310915*cos(q1L))/9007199254740992 + (5557241208790345*sin(q1L))/9007199254740992))/332306998946228968225951765070086144 + (9007199067919185*sin(q2L)*((5557241208790345*cos(q1L))/9007199254740992 - (6384186990310915*sin(q1L))/9007199254740992))/9007199254740992 - 347859890694807798813742879236295256254610072729/24519928653854221733733552434404946937899825954937634816)))/36893488147419103232000 + (712008244765680093343103025701132101054572137019*sin(q5L)*((7514214926474921*cos(q4L)*((7514214926474921*cos(q3L)*((55491554575214198102159220722265*cos(q2L))/162259276829213363391578010288128 + (7514214926474921*cos(q2L)*((6384186990310915*cos(q1L))/9007199254740992 + (5557241208790345*sin(q1L))/9007199254740992))/36893488147419103232 - sin(q2L)*((5557241208790345*cos(q1L))/9007199254740992 - (6384186990310915*sin(q1L))/9007199254740992)))/36893488147419103232 + (9007199067919185*cos(q3L)*((57503643108550260546605243404275*cos(q1L))/81129638414606681695789005144064 + (50055177836018480443110068268825*sin(q1L))/81129638414606681695789005144064 - 46293577452674263141823442369649/664613997892457936451903530140172288))/9007199254740992 + sin(q3L)*((55491554575214198102159220722265*sin(q2L))/162259276829213363391578010288128 + cos(q2L)*((5557241208790345*cos(q1L))/9007199254740992 - (6384186990310915*sin(q1L))/9007199254740992) + (7514214926474921*sin(q2L)*((6384186990310915*cos(q1L))/9007199254740992 + (5557241208790345*sin(q1L))/9007199254740992))/36893488147419103232)))/36893488147419103232 + ((4503599440548691*cos(q4L))/4503599627370496 - (7514214926474921*sin(q4L))/36893488147419103232)*((7514214926474921*sin(q3L)*((55491554575214198102159220722265*cos(q2L))/162259276829213363391578010288128 + (7514214926474921*cos(q2L)*((6384186990310915*cos(q1L))/9007199254740992 + (5557241208790345*sin(q1L))/9007199254740992))/36893488147419103232 - sin(q2L)*((5557241208790345*cos(q1L))/9007199254740992 - (6384186990310915*sin(q1L))/9007199254740992)))/36893488147419103232 - cos(q3L)*((55491554575214198102159220722265*sin(q2L))/162259276829213363391578010288128 + cos(q2L)*((5557241208790345*cos(q1L))/9007199254740992 - (6384186990310915*sin(q1L))/9007199254740992) + (7514214926474921*sin(q2L)*((6384186990310915*cos(q1L))/9007199254740992 + (5557241208790345*sin(q1L))/9007199254740992))/36893488147419103232) + (9007199067919185*sin(q3L)*((57503643108550260546605243404275*cos(q1L))/81129638414606681695789005144064 + (50055177836018480443110068268825*sin(q1L))/81129638414606681695789005144064 - 46293577452674263141823442369649/664613997892457936451903530140172288))/9007199254740992) + ((234819211581865*cos(q4L))/1152921504606846976 + (9007199067919185*sin(q4L))/9007199254740992)*((432094733372955093709245836907320566011451687275*cos(q1L))/2993155353253689176481146537402947624255349848014848 - (499823478647255911063139966257565597426350154025*cos(q2L))/1461501637330902918203684832716283019655932542976 + (376125364442766701270516501597006072214248637825*sin(q1L))/2993155353253689176481146537402947624255349848014848 - (67682029681889335677290557259385*cos(q2L)*((6384186990310915*cos(q1L))/9007199254740992 + (5557241208790345*sin(q1L))/9007199254740992))/332306998946228968225951765070086144 + (9007199067919185*sin(q2L)*((5557241208790345*cos(q1L))/9007199254740992 - (6384186990310915*sin(q1L))/9007199254740992))/9007199254740992 - 347859890694807798813742879236295256254610072729/24519928653854221733733552434404946937899825954937634816)))/2451992865385422173373355243440494693789982595493763481600 - (94754841554645069948206780163139*cos(q5L)*((7514214926474921*sin(q4L)*((7514214926474921*cos(q3L)*((55491554575214198102159220722265*cos(q2L))/162259276829213363391578010288128 + (7514214926474921*cos(q2L)*((6384186990310915*cos(q1L))/9007199254740992 + (5557241208790345*sin(q1L))/9007199254740992))/36893488147419103232 - sin(q2L)*((5557241208790345*cos(q1L))/9007199254740992 - (6384186990310915*sin(q1L))/9007199254740992)))/36893488147419103232 + (9007199067919185*cos(q3L)*((57503643108550260546605243404275*cos(q1L))/81129638414606681695789005144064 + (50055177836018480443110068268825*sin(q1L))/81129638414606681695789005144064 - 46293577452674263141823442369649/664613997892457936451903530140172288))/9007199254740992 + sin(q3L)*((55491554575214198102159220722265*sin(q2L))/162259276829213363391578010288128 + cos(q2L)*((5557241208790345*cos(q1L))/9007199254740992 - (6384186990310915*sin(q1L))/9007199254740992) + (7514214926474921*sin(q2L)*((6384186990310915*cos(q1L))/9007199254740992 + (5557241208790345*sin(q1L))/9007199254740992))/36893488147419103232)))/36893488147419103232 + ((7514214926474921*cos(q4L))/36893488147419103232 + (4503599440548691*sin(q4L))/4503599627370496)*((7514214926474921*sin(q3L)*((55491554575214198102159220722265*cos(q2L))/162259276829213363391578010288128 + (7514214926474921*cos(q2L)*((6384186990310915*cos(q1L))/9007199254740992 + (5557241208790345*sin(q1L))/9007199254740992))/36893488147419103232 - sin(q2L)*((5557241208790345*cos(q1L))/9007199254740992 - (6384186990310915*sin(q1L))/9007199254740992)))/36893488147419103232 - cos(q3L)*((55491554575214198102159220722265*sin(q2L))/162259276829213363391578010288128 + cos(q2L)*((5557241208790345*cos(q1L))/9007199254740992 - (6384186990310915*sin(q1L))/9007199254740992) + (7514214926474921*sin(q2L)*((6384186990310915*cos(q1L))/9007199254740992 + (5557241208790345*sin(q1L))/9007199254740992))/36893488147419103232) + (9007199067919185*sin(q3L)*((57503643108550260546605243404275*cos(q1L))/81129638414606681695789005144064 + (50055177836018480443110068268825*sin(q1L))/81129638414606681695789005144064 - 46293577452674263141823442369649/664613997892457936451903530140172288))/9007199254740992) - ((9007199067919185*cos(q4L))/9007199254740992 - (234819211581865*sin(q4L))/1152921504606846976)*((432094733372955093709245836907320566011451687275*cos(q1L))/2993155353253689176481146537402947624255349848014848 - (499823478647255911063139966257565597426350154025*cos(q2L))/1461501637330902918203684832716283019655932542976 + (376125364442766701270516501597006072214248637825*sin(q1L))/2993155353253689176481146537402947624255349848014848 - (67682029681889335677290557259385*cos(q2L)*((6384186990310915*cos(q1L))/9007199254740992 + (5557241208790345*sin(q1L))/9007199254740992))/332306998946228968225951765070086144 + (9007199067919185*sin(q2L)*((5557241208790345*cos(q1L))/9007199254740992 - (6384186990310915*sin(q1L))/9007199254740992))/9007199254740992 - 347859890694807798813742879236295256254610072729/24519928653854221733733552434404946937899825954937634816)))/66461399789245793645190353014017228800 + (27*sin(q5L)*((7514214926474921*sin(q4L)*((7514214926474921*cos(q3L)*((55491554575214198102159220722265*cos(q2L))/162259276829213363391578010288128 + (7514214926474921*cos(q2L)*((6384186990310915*cos(q1L))/9007199254740992 + (5557241208790345*sin(q1L))/9007199254740992))/36893488147419103232 - sin(q2L)*((5557241208790345*cos(q1L))/9007199254740992 - (6384186990310915*sin(q1L))/9007199254740992)))/36893488147419103232 + (9007199067919185*cos(q3L)*((57503643108550260546605243404275*cos(q1L))/81129638414606681695789005144064 + (50055177836018480443110068268825*sin(q1L))/81129638414606681695789005144064 - 46293577452674263141823442369649/664613997892457936451903530140172288))/9007199254740992 + sin(q3L)*((55491554575214198102159220722265*sin(q2L))/162259276829213363391578010288128 + cos(q2L)*((5557241208790345*cos(q1L))/9007199254740992 - (6384186990310915*sin(q1L))/9007199254740992) + (7514214926474921*sin(q2L)*((6384186990310915*cos(q1L))/9007199254740992 + (5557241208790345*sin(q1L))/9007199254740992))/36893488147419103232)))/36893488147419103232 + ((7514214926474921*cos(q4L))/36893488147419103232 + (4503599440548691*sin(q4L))/4503599627370496)*((7514214926474921*sin(q3L)*((55491554575214198102159220722265*cos(q2L))/162259276829213363391578010288128 + (7514214926474921*cos(q2L)*((6384186990310915*cos(q1L))/9007199254740992 + (5557241208790345*sin(q1L))/9007199254740992))/36893488147419103232 - sin(q2L)*((5557241208790345*cos(q1L))/9007199254740992 - (6384186990310915*sin(q1L))/9007199254740992)))/36893488147419103232 - cos(q3L)*((55491554575214198102159220722265*sin(q2L))/162259276829213363391578010288128 + cos(q2L)*((5557241208790345*cos(q1L))/9007199254740992 - (6384186990310915*sin(q1L))/9007199254740992) + (7514214926474921*sin(q2L)*((6384186990310915*cos(q1L))/9007199254740992 + (5557241208790345*sin(q1L))/9007199254740992))/36893488147419103232) + (9007199067919185*sin(q3L)*((57503643108550260546605243404275*cos(q1L))/81129638414606681695789005144064 + (50055177836018480443110068268825*sin(q1L))/81129638414606681695789005144064 - 46293577452674263141823442369649/664613997892457936451903530140172288))/9007199254740992) - ((9007199067919185*cos(q4L))/9007199254740992 - (234819211581865*sin(q4L))/1152921504606846976)*((432094733372955093709245836907320566011451687275*cos(q1L))/2993155353253689176481146537402947624255349848014848 - (499823478647255911063139966257565597426350154025*cos(q2L))/1461501637330902918203684832716283019655932542976 + (376125364442766701270516501597006072214248637825*sin(q1L))/2993155353253689176481146537402947624255349848014848 - (67682029681889335677290557259385*cos(q2L)*((6384186990310915*cos(q1L))/9007199254740992 + (5557241208790345*sin(q1L))/9007199254740992))/332306998946228968225951765070086144 + (9007199067919185*sin(q2L)*((5557241208790345*cos(q1L))/9007199254740992 - (6384186990310915*sin(q1L))/9007199254740992))/9007199254740992 - 347859890694807798813742879236295256254610072729/24519928653854221733733552434404946937899825954937634816)))/1000, (202883803014822867*cos(q6L)*((9007199067919185*cos(q5L)*((783310804561232573774573497517025067305577458842146606386579375*cos(q2L))/55213970774324510299478046898216203619608871777363092441300193790394368 - (677168015718420743488926864722853474412798830140650728756148125*cos(q1L))/113078212145816597093331040047546785012958969400039613319782796882727665664 - (589454226189876320500100500762517606499114263738369612804244375*sin(q1L))/113078212145816597093331040047546785012958969400039613319782796882727665664 + (106069577339469832923929692356850887620017617375*cos(q2L)*((6384186990310915*cos(q1L))/9007199254740992 + (5557241208790345*sin(q1L))/9007199254740992))/12554203470773361527671578846415332832204710888928069025792 - (14115856197532180673579726082375*sin(q2L)*((5557241208790345*cos(q1L))/9007199254740992 - (6384186990310915*sin(q1L))/9007199254740992))/340282366920938463463374607431768211456 + (67682029681889335677290557259385*cos(q3L)*((55491554575214198102159220722265*cos(q2L))/162259276829213363391578010288128 + (7514214926474921*cos(q2L)*((6384186990310915*cos(q1L))/9007199254740992 + (5557241208790345*sin(q1L))/9007199254740992))/36893488147419103232 - sin(q2L)*((5557241208790345*cos(q1L))/9007199254740992 - (6384186990310915*sin(q1L))/9007199254740992)))/332306998946228968225951765070086144 + (234819211581865*cos(q3L)*((55491554575214198102159220722265*sin(q2L))/162259276829213363391578010288128 + cos(q2L)*((5557241208790345*cos(q1L))/9007199254740992 - (6384186990310915*sin(q1L))/9007199254740992) + (7514214926474921*sin(q2L)*((6384186990310915*cos(q1L))/9007199254740992 + (5557241208790345*sin(q1L))/9007199254740992))/36893488147419103232))/1152921504606846976 - (1764482024691522628700660907665*sin(q3L)*((55491554575214198102159220722265*cos(q2L))/162259276829213363391578010288128 + (7514214926474921*cos(q2L)*((6384186990310915*cos(q1L))/9007199254740992 + (5557241208790345*sin(q1L))/9007199254740992))/36893488147419103232 - sin(q2L)*((5557241208790345*cos(q1L))/9007199254740992 - (6384186990310915*sin(q1L))/9007199254740992)))/42535295865117307932921825928971026432 + (81129635049124235038645691064225*cos(q3L)*((57503643108550260546605243404275*cos(q1L))/81129638414606681695789005144064 + (50055177836018480443110068268825*sin(q1L))/81129638414606681695789005144064 - 46293577452674263141823442369649/664613997892457936451903530140172288))/81129638414606681695789005144064 + (9007199067919185*sin(q3L)*((55491554575214198102159220722265*sin(q2L))/162259276829213363391578010288128 + cos(q2L)*((5557241208790345*cos(q1L))/9007199254740992 - (6384186990310915*sin(q1L))/9007199254740992) + (7514214926474921*sin(q2L)*((6384186990310915*cos(q1L))/9007199254740992 + (5557241208790345*sin(q1L))/9007199254740992))/36893488147419103232))/9007199254740992 - (2115063383689692319117831580025*sin(q3L)*((57503643108550260546605243404275*cos(q1L))/81129638414606681695789005144064 + (50055177836018480443110068268825*sin(q1L))/81129638414606681695789005144064 - 46293577452674263141823442369649/664613997892457936451903530140172288))/10384593717069655257060992658440192 + 545157285512458543963749743061519108960107968042455893206992575/926336713898529563388567880069503262826159877325124512315660672063305037119488))/9007199254740992 + (7514214926474921*cos(q5L)*((7514214926474921*cos(q4L)*((7514214926474921*cos(q3L)*((55491554575214198102159220722265*cos(q2L))/162259276829213363391578010288128 + (7514214926474921*cos(q2L)*((6384186990310915*cos(q1L))/9007199254740992 + (5557241208790345*sin(q1L))/9007199254740992))/36893488147419103232 - sin(q2L)*((5557241208790345*cos(q1L))/9007199254740992 - (6384186990310915*sin(q1L))/9007199254740992)))/36893488147419103232 + (9007199067919185*cos(q3L)*((57503643108550260546605243404275*cos(q1L))/81129638414606681695789005144064 + (50055177836018480443110068268825*sin(q1L))/81129638414606681695789005144064 - 46293577452674263141823442369649/664613997892457936451903530140172288))/9007199254740992 + sin(q3L)*((55491554575214198102159220722265*sin(q2L))/162259276829213363391578010288128 + cos(q2L)*((5557241208790345*cos(q1L))/9007199254740992 - (6384186990310915*sin(q1L))/9007199254740992) + (7514214926474921*sin(q2L)*((6384186990310915*cos(q1L))/9007199254740992 + (5557241208790345*sin(q1L))/9007199254740992))/36893488147419103232)))/36893488147419103232 + ((4503599440548691*cos(q4L))/4503599627370496 - (7514214926474921*sin(q4L))/36893488147419103232)*((7514214926474921*sin(q3L)*((55491554575214198102159220722265*cos(q2L))/162259276829213363391578010288128 + (7514214926474921*cos(q2L)*((6384186990310915*cos(q1L))/9007199254740992 + (5557241208790345*sin(q1L))/9007199254740992))/36893488147419103232 - sin(q2L)*((5557241208790345*cos(q1L))/9007199254740992 - (6384186990310915*sin(q1L))/9007199254740992)))/36893488147419103232 - cos(q3L)*((55491554575214198102159220722265*sin(q2L))/162259276829213363391578010288128 + cos(q2L)*((5557241208790345*cos(q1L))/9007199254740992 - (6384186990310915*sin(q1L))/9007199254740992) + (7514214926474921*sin(q2L)*((6384186990310915*cos(q1L))/9007199254740992 + (5557241208790345*sin(q1L))/9007199254740992))/36893488147419103232) + (9007199067919185*sin(q3L)*((57503643108550260546605243404275*cos(q1L))/81129638414606681695789005144064 + (50055177836018480443110068268825*sin(q1L))/81129638414606681695789005144064 - 46293577452674263141823442369649/664613997892457936451903530140172288))/9007199254740992) + ((234819211581865*cos(q4L))/1152921504606846976 + (9007199067919185*sin(q4L))/9007199254740992)*((432094733372955093709245836907320566011451687275*cos(q1L))/2993155353253689176481146537402947624255349848014848 - (499823478647255911063139966257565597426350154025*cos(q2L))/1461501637330902918203684832716283019655932542976 + (376125364442766701270516501597006072214248637825*sin(q1L))/2993155353253689176481146537402947624255349848014848 - (67682029681889335677290557259385*cos(q2L)*((6384186990310915*cos(q1L))/9007199254740992 + (5557241208790345*sin(q1L))/9007199254740992))/332306998946228968225951765070086144 + (9007199067919185*sin(q2L)*((5557241208790345*cos(q1L))/9007199254740992 - (6384186990310915*sin(q1L))/9007199254740992))/9007199254740992 - 347859890694807798813742879236295256254610072729/24519928653854221733733552434404946937899825954937634816)))/36893488147419103232 + sin(q5L)*((7514214926474921*sin(q4L)*((7514214926474921*cos(q3L)*((55491554575214198102159220722265*cos(q2L))/162259276829213363391578010288128 + (7514214926474921*cos(q2L)*((6384186990310915*cos(q1L))/9007199254740992 + (5557241208790345*sin(q1L))/9007199254740992))/36893488147419103232 - sin(q2L)*((5557241208790345*cos(q1L))/9007199254740992 - (6384186990310915*sin(q1L))/9007199254740992)))/36893488147419103232 + (9007199067919185*cos(q3L)*((57503643108550260546605243404275*cos(q1L))/81129638414606681695789005144064 + (50055177836018480443110068268825*sin(q1L))/81129638414606681695789005144064 - 46293577452674263141823442369649/664613997892457936451903530140172288))/9007199254740992 + sin(q3L)*((55491554575214198102159220722265*sin(q2L))/162259276829213363391578010288128 + cos(q2L)*((5557241208790345*cos(q1L))/9007199254740992 - (6384186990310915*sin(q1L))/9007199254740992) + (7514214926474921*sin(q2L)*((6384186990310915*cos(q1L))/9007199254740992 + (5557241208790345*sin(q1L))/9007199254740992))/36893488147419103232)))/36893488147419103232 + ((7514214926474921*cos(q4L))/36893488147419103232 + (4503599440548691*sin(q4L))/4503599627370496)*((7514214926474921*sin(q3L)*((55491554575214198102159220722265*cos(q2L))/162259276829213363391578010288128 + (7514214926474921*cos(q2L)*((6384186990310915*cos(q1L))/9007199254740992 + (5557241208790345*sin(q1L))/9007199254740992))/36893488147419103232 - sin(q2L)*((5557241208790345*cos(q1L))/9007199254740992 - (6384186990310915*sin(q1L))/9007199254740992)))/36893488147419103232 - cos(q3L)*((55491554575214198102159220722265*sin(q2L))/162259276829213363391578010288128 + cos(q2L)*((5557241208790345*cos(q1L))/9007199254740992 - (6384186990310915*sin(q1L))/9007199254740992) + (7514214926474921*sin(q2L)*((6384186990310915*cos(q1L))/9007199254740992 + (5557241208790345*sin(q1L))/9007199254740992))/36893488147419103232) + (9007199067919185*sin(q3L)*((57503643108550260546605243404275*cos(q1L))/81129638414606681695789005144064 + (50055177836018480443110068268825*sin(q1L))/81129638414606681695789005144064 - 46293577452674263141823442369649/664613997892457936451903530140172288))/9007199254740992) - ((9007199067919185*cos(q4L))/9007199254740992 - (234819211581865*sin(q4L))/1152921504606846976)*((432094733372955093709245836907320566011451687275*cos(q1L))/2993155353253689176481146537402947624255349848014848 - (499823478647255911063139966257565597426350154025*cos(q2L))/1461501637330902918203684832716283019655932542976 + (376125364442766701270516501597006072214248637825*sin(q1L))/2993155353253689176481146537402947624255349848014848 - (67682029681889335677290557259385*cos(q2L)*((6384186990310915*cos(q1L))/9007199254740992 + (5557241208790345*sin(q1L))/9007199254740992))/332306998946228968225951765070086144 + (9007199067919185*sin(q2L)*((5557241208790345*cos(q1L))/9007199254740992 - (6384186990310915*sin(q1L))/9007199254740992))/9007199254740992 - 347859890694807798813742879236295256254610072729/24519928653854221733733552434404946937899825954937634816))))/36893488147419103232000 - (2436553109258773196144549622003023*sin(q6L)*((9007199067919185*cos(q5L)*((783310804561232573774573497517025067305577458842146606386579375*cos(q2L))/55213970774324510299478046898216203619608871777363092441300193790394368 - (677168015718420743488926864722853474412798830140650728756148125*cos(q1L))/113078212145816597093331040047546785012958969400039613319782796882727665664 - (589454226189876320500100500762517606499114263738369612804244375*sin(q1L))/113078212145816597093331040047546785012958969400039613319782796882727665664 + (106069577339469832923929692356850887620017617375*cos(q2L)*((6384186990310915*cos(q1L))/9007199254740992 + (5557241208790345*sin(q1L))/9007199254740992))/12554203470773361527671578846415332832204710888928069025792 - (14115856197532180673579726082375*sin(q2L)*((5557241208790345*cos(q1L))/9007199254740992 - (6384186990310915*sin(q1L))/9007199254740992))/340282366920938463463374607431768211456 + (67682029681889335677290557259385*cos(q3L)*((55491554575214198102159220722265*cos(q2L))/162259276829213363391578010288128 + (7514214926474921*cos(q2L)*((6384186990310915*cos(q1L))/9007199254740992 + (5557241208790345*sin(q1L))/9007199254740992))/36893488147419103232 - sin(q2L)*((5557241208790345*cos(q1L))/9007199254740992 - (6384186990310915*sin(q1L))/9007199254740992)))/332306998946228968225951765070086144 + (234819211581865*cos(q3L)*((55491554575214198102159220722265*sin(q2L))/162259276829213363391578010288128 + cos(q2L)*((5557241208790345*cos(q1L))/9007199254740992 - (6384186990310915*sin(q1L))/9007199254740992) + (7514214926474921*sin(q2L)*((6384186990310915*cos(q1L))/9007199254740992 + (5557241208790345*sin(q1L))/9007199254740992))/36893488147419103232))/1152921504606846976 - (1764482024691522628700660907665*sin(q3L)*((55491554575214198102159220722265*cos(q2L))/162259276829213363391578010288128 + (7514214926474921*cos(q2L)*((6384186990310915*cos(q1L))/9007199254740992 + (5557241208790345*sin(q1L))/9007199254740992))/36893488147419103232 - sin(q2L)*((5557241208790345*cos(q1L))/9007199254740992 - (6384186990310915*sin(q1L))/9007199254740992)))/42535295865117307932921825928971026432 + (81129635049124235038645691064225*cos(q3L)*((57503643108550260546605243404275*cos(q1L))/81129638414606681695789005144064 + (50055177836018480443110068268825*sin(q1L))/81129638414606681695789005144064 - 46293577452674263141823442369649/664613997892457936451903530140172288))/81129638414606681695789005144064 + (9007199067919185*sin(q3L)*((55491554575214198102159220722265*sin(q2L))/162259276829213363391578010288128 + cos(q2L)*((5557241208790345*cos(q1L))/9007199254740992 - (6384186990310915*sin(q1L))/9007199254740992) + (7514214926474921*sin(q2L)*((6384186990310915*cos(q1L))/9007199254740992 + (5557241208790345*sin(q1L))/9007199254740992))/36893488147419103232))/9007199254740992 - (2115063383689692319117831580025*sin(q3L)*((57503643108550260546605243404275*cos(q1L))/81129638414606681695789005144064 + (50055177836018480443110068268825*sin(q1L))/81129638414606681695789005144064 - 46293577452674263141823442369649/664613997892457936451903530140172288))/10384593717069655257060992658440192 + 545157285512458543963749743061519108960107968042455893206992575/926336713898529563388567880069503262826159877325124512315660672063305037119488))/9007199254740992 + (7514214926474921*cos(q5L)*((7514214926474921*cos(q4L)*((7514214926474921*cos(q3L)*((55491554575214198102159220722265*cos(q2L))/162259276829213363391578010288128 + (7514214926474921*cos(q2L)*((6384186990310915*cos(q1L))/9007199254740992 + (5557241208790345*sin(q1L))/9007199254740992))/36893488147419103232 - sin(q2L)*((5557241208790345*cos(q1L))/9007199254740992 - (6384186990310915*sin(q1L))/9007199254740992)))/36893488147419103232 + (9007199067919185*cos(q3L)*((57503643108550260546605243404275*cos(q1L))/81129638414606681695789005144064 + (50055177836018480443110068268825*sin(q1L))/81129638414606681695789005144064 - 46293577452674263141823442369649/664613997892457936451903530140172288))/9007199254740992 + sin(q3L)*((55491554575214198102159220722265*sin(q2L))/162259276829213363391578010288128 + cos(q2L)*((5557241208790345*cos(q1L))/9007199254740992 - (6384186990310915*sin(q1L))/9007199254740992) + (7514214926474921*sin(q2L)*((6384186990310915*cos(q1L))/9007199254740992 + (5557241208790345*sin(q1L))/9007199254740992))/36893488147419103232)))/36893488147419103232 + ((4503599440548691*cos(q4L))/4503599627370496 - (7514214926474921*sin(q4L))/36893488147419103232)*((7514214926474921*sin(q3L)*((55491554575214198102159220722265*cos(q2L))/162259276829213363391578010288128 + (7514214926474921*cos(q2L)*((6384186990310915*cos(q1L))/9007199254740992 + (5557241208790345*sin(q1L))/9007199254740992))/36893488147419103232 - sin(q2L)*((5557241208790345*cos(q1L))/9007199254740992 - (6384186990310915*sin(q1L))/9007199254740992)))/36893488147419103232 - cos(q3L)*((55491554575214198102159220722265*sin(q2L))/162259276829213363391578010288128 + cos(q2L)*((5557241208790345*cos(q1L))/9007199254740992 - (6384186990310915*sin(q1L))/9007199254740992) + (7514214926474921*sin(q2L)*((6384186990310915*cos(q1L))/9007199254740992 + (5557241208790345*sin(q1L))/9007199254740992))/36893488147419103232) + (9007199067919185*sin(q3L)*((57503643108550260546605243404275*cos(q1L))/81129638414606681695789005144064 + (50055177836018480443110068268825*sin(q1L))/81129638414606681695789005144064 - 46293577452674263141823442369649/664613997892457936451903530140172288))/9007199254740992) + ((234819211581865*cos(q4L))/1152921504606846976 + (9007199067919185*sin(q4L))/9007199254740992)*((432094733372955093709245836907320566011451687275*cos(q1L))/2993155353253689176481146537402947624255349848014848 - (499823478647255911063139966257565597426350154025*cos(q2L))/1461501637330902918203684832716283019655932542976 + (376125364442766701270516501597006072214248637825*sin(q1L))/2993155353253689176481146537402947624255349848014848 - (67682029681889335677290557259385*cos(q2L)*((6384186990310915*cos(q1L))/9007199254740992 + (5557241208790345*sin(q1L))/9007199254740992))/332306998946228968225951765070086144 + (9007199067919185*sin(q2L)*((5557241208790345*cos(q1L))/9007199254740992 - (6384186990310915*sin(q1L))/9007199254740992))/9007199254740992 - 347859890694807798813742879236295256254610072729/24519928653854221733733552434404946937899825954937634816)))/36893488147419103232 + sin(q5L)*((7514214926474921*sin(q4L)*((7514214926474921*cos(q3L)*((55491554575214198102159220722265*cos(q2L))/162259276829213363391578010288128 + (7514214926474921*cos(q2L)*((6384186990310915*cos(q1L))/9007199254740992 + (5557241208790345*sin(q1L))/9007199254740992))/36893488147419103232 - sin(q2L)*((5557241208790345*cos(q1L))/9007199254740992 - (6384186990310915*sin(q1L))/9007199254740992)))/36893488147419103232 + (9007199067919185*cos(q3L)*((57503643108550260546605243404275*cos(q1L))/81129638414606681695789005144064 + (50055177836018480443110068268825*sin(q1L))/81129638414606681695789005144064 - 46293577452674263141823442369649/664613997892457936451903530140172288))/9007199254740992 + sin(q3L)*((55491554575214198102159220722265*sin(q2L))/162259276829213363391578010288128 + cos(q2L)*((5557241208790345*cos(q1L))/9007199254740992 - (6384186990310915*sin(q1L))/9007199254740992) + (7514214926474921*sin(q2L)*((6384186990310915*cos(q1L))/9007199254740992 + (5557241208790345*sin(q1L))/9007199254740992))/36893488147419103232)))/36893488147419103232 + ((7514214926474921*cos(q4L))/36893488147419103232 + (4503599440548691*sin(q4L))/4503599627370496)*((7514214926474921*sin(q3L)*((55491554575214198102159220722265*cos(q2L))/162259276829213363391578010288128 + (7514214926474921*cos(q2L)*((6384186990310915*cos(q1L))/9007199254740992 + (5557241208790345*sin(q1L))/9007199254740992))/36893488147419103232 - sin(q2L)*((5557241208790345*cos(q1L))/9007199254740992 - (6384186990310915*sin(q1L))/9007199254740992)))/36893488147419103232 - cos(q3L)*((55491554575214198102159220722265*sin(q2L))/162259276829213363391578010288128 + cos(q2L)*((5557241208790345*cos(q1L))/9007199254740992 - (6384186990310915*sin(q1L))/9007199254740992) + (7514214926474921*sin(q2L)*((6384186990310915*cos(q1L))/9007199254740992 + (5557241208790345*sin(q1L))/9007199254740992))/36893488147419103232) + (9007199067919185*sin(q3L)*((57503643108550260546605243404275*cos(q1L))/81129638414606681695789005144064 + (50055177836018480443110068268825*sin(q1L))/81129638414606681695789005144064 - 46293577452674263141823442369649/664613997892457936451903530140172288))/9007199254740992) - ((9007199067919185*cos(q4L))/9007199254740992 - (234819211581865*sin(q4L))/1152921504606846976)*((432094733372955093709245836907320566011451687275*cos(q1L))/2993155353253689176481146537402947624255349848014848 - (499823478647255911063139966257565597426350154025*cos(q2L))/1461501637330902918203684832716283019655932542976 + (376125364442766701270516501597006072214248637825*sin(q1L))/2993155353253689176481146537402947624255349848014848 - (67682029681889335677290557259385*cos(q2L)*((6384186990310915*cos(q1L))/9007199254740992 + (5557241208790345*sin(q1L))/9007199254740992))/332306998946228968225951765070086144 + (9007199067919185*sin(q2L)*((5557241208790345*cos(q1L))/9007199254740992 - (6384186990310915*sin(q1L))/9007199254740992))/9007199254740992 - 347859890694807798813742879236295256254610072729/24519928653854221733733552434404946937899825954937634816))))/332306998946228968225951765070086144000 + (324259171862923063*cos(q6L)*((9007199067919185*sin(q5L)*((783310804561232573774573497517025067305577458842146606386579375*cos(q2L))/55213970774324510299478046898216203619608871777363092441300193790394368 - (677168015718420743488926864722853474412798830140650728756148125*cos(q1L))/113078212145816597093331040047546785012958969400039613319782796882727665664 - (589454226189876320500100500762517606499114263738369612804244375*sin(q1L))/113078212145816597093331040047546785012958969400039613319782796882727665664 + (106069577339469832923929692356850887620017617375*cos(q2L)*((6384186990310915*cos(q1L))/9007199254740992 + (5557241208790345*sin(q1L))/9007199254740992))/12554203470773361527671578846415332832204710888928069025792 - (14115856197532180673579726082375*sin(q2L)*((5557241208790345*cos(q1L))/9007199254740992 - (6384186990310915*sin(q1L))/9007199254740992))/340282366920938463463374607431768211456 + (67682029681889335677290557259385*cos(q3L)*((55491554575214198102159220722265*cos(q2L))/162259276829213363391578010288128 + (7514214926474921*cos(q2L)*((6384186990310915*cos(q1L))/9007199254740992 + (5557241208790345*sin(q1L))/9007199254740992))/36893488147419103232 - sin(q2L)*((5557241208790345*cos(q1L))/9007199254740992 - (6384186990310915*sin(q1L))/9007199254740992)))/332306998946228968225951765070086144 + (234819211581865*cos(q3L)*((55491554575214198102159220722265*sin(q2L))/162259276829213363391578010288128 + cos(q2L)*((5557241208790345*cos(q1L))/9007199254740992 - (6384186990310915*sin(q1L))/9007199254740992) + (7514214926474921*sin(q2L)*((6384186990310915*cos(q1L))/9007199254740992 + (5557241208790345*sin(q1L))/9007199254740992))/36893488147419103232))/1152921504606846976 - (1764482024691522628700660907665*sin(q3L)*((55491554575214198102159220722265*cos(q2L))/162259276829213363391578010288128 + (7514214926474921*cos(q2L)*((6384186990310915*cos(q1L))/9007199254740992 + (5557241208790345*sin(q1L))/9007199254740992))/36893488147419103232 - sin(q2L)*((5557241208790345*cos(q1L))/9007199254740992 - (6384186990310915*sin(q1L))/9007199254740992)))/42535295865117307932921825928971026432 + (81129635049124235038645691064225*cos(q3L)*((57503643108550260546605243404275*cos(q1L))/81129638414606681695789005144064 + (50055177836018480443110068268825*sin(q1L))/81129638414606681695789005144064 - 46293577452674263141823442369649/664613997892457936451903530140172288))/81129638414606681695789005144064 + (9007199067919185*sin(q3L)*((55491554575214198102159220722265*sin(q2L))/162259276829213363391578010288128 + cos(q2L)*((5557241208790345*cos(q1L))/9007199254740992 - (6384186990310915*sin(q1L))/9007199254740992) + (7514214926474921*sin(q2L)*((6384186990310915*cos(q1L))/9007199254740992 + (5557241208790345*sin(q1L))/9007199254740992))/36893488147419103232))/9007199254740992 - (2115063383689692319117831580025*sin(q3L)*((57503643108550260546605243404275*cos(q1L))/81129638414606681695789005144064 + (50055177836018480443110068268825*sin(q1L))/81129638414606681695789005144064 - 46293577452674263141823442369649/664613997892457936451903530140172288))/10384593717069655257060992658440192 + 545157285512458543963749743061519108960107968042455893206992575/926336713898529563388567880069503262826159877325124512315660672063305037119488))/9007199254740992 + (7514214926474921*sin(q5L)*((7514214926474921*cos(q4L)*((7514214926474921*cos(q3L)*((55491554575214198102159220722265*cos(q2L))/162259276829213363391578010288128 + (7514214926474921*cos(q2L)*((6384186990310915*cos(q1L))/9007199254740992 + (5557241208790345*sin(q1L))/9007199254740992))/36893488147419103232 - sin(q2L)*((5557241208790345*cos(q1L))/9007199254740992 - (6384186990310915*sin(q1L))/9007199254740992)))/36893488147419103232 + (9007199067919185*cos(q3L)*((57503643108550260546605243404275*cos(q1L))/81129638414606681695789005144064 + (50055177836018480443110068268825*sin(q1L))/81129638414606681695789005144064 - 46293577452674263141823442369649/664613997892457936451903530140172288))/9007199254740992 + sin(q3L)*((55491554575214198102159220722265*sin(q2L))/162259276829213363391578010288128 + cos(q2L)*((5557241208790345*cos(q1L))/9007199254740992 - (6384186990310915*sin(q1L))/9007199254740992) + (7514214926474921*sin(q2L)*((6384186990310915*cos(q1L))/9007199254740992 + (5557241208790345*sin(q1L))/9007199254740992))/36893488147419103232)))/36893488147419103232 + ((4503599440548691*cos(q4L))/4503599627370496 - (7514214926474921*sin(q4L))/36893488147419103232)*((7514214926474921*sin(q3L)*((55491554575214198102159220722265*cos(q2L))/162259276829213363391578010288128 + (7514214926474921*cos(q2L)*((6384186990310915*cos(q1L))/9007199254740992 + (5557241208790345*sin(q1L))/9007199254740992))/36893488147419103232 - sin(q2L)*((5557241208790345*cos(q1L))/9007199254740992 - (6384186990310915*sin(q1L))/9007199254740992)))/36893488147419103232 - cos(q3L)*((55491554575214198102159220722265*sin(q2L))/162259276829213363391578010288128 + cos(q2L)*((5557241208790345*cos(q1L))/9007199254740992 - (6384186990310915*sin(q1L))/9007199254740992) + (7514214926474921*sin(q2L)*((6384186990310915*cos(q1L))/9007199254740992 + (5557241208790345*sin(q1L))/9007199254740992))/36893488147419103232) + (9007199067919185*sin(q3L)*((57503643108550260546605243404275*cos(q1L))/81129638414606681695789005144064 + (50055177836018480443110068268825*sin(q1L))/81129638414606681695789005144064 - 46293577452674263141823442369649/664613997892457936451903530140172288))/9007199254740992) + ((234819211581865*cos(q4L))/1152921504606846976 + (9007199067919185*sin(q4L))/9007199254740992)*((432094733372955093709245836907320566011451687275*cos(q1L))/2993155353253689176481146537402947624255349848014848 - (499823478647255911063139966257565597426350154025*cos(q2L))/1461501637330902918203684832716283019655932542976 + (376125364442766701270516501597006072214248637825*sin(q1L))/2993155353253689176481146537402947624255349848014848 - (67682029681889335677290557259385*cos(q2L)*((6384186990310915*cos(q1L))/9007199254740992 + (5557241208790345*sin(q1L))/9007199254740992))/332306998946228968225951765070086144 + (9007199067919185*sin(q2L)*((5557241208790345*cos(q1L))/9007199254740992 - (6384186990310915*sin(q1L))/9007199254740992))/9007199254740992 - 347859890694807798813742879236295256254610072729/24519928653854221733733552434404946937899825954937634816)))/36893488147419103232 - cos(q5L)*((7514214926474921*sin(q4L)*((7514214926474921*cos(q3L)*((55491554575214198102159220722265*cos(q2L))/162259276829213363391578010288128 + (7514214926474921*cos(q2L)*((6384186990310915*cos(q1L))/9007199254740992 + (5557241208790345*sin(q1L))/9007199254740992))/36893488147419103232 - sin(q2L)*((5557241208790345*cos(q1L))/9007199254740992 - (6384186990310915*sin(q1L))/9007199254740992)))/36893488147419103232 + (9007199067919185*cos(q3L)*((57503643108550260546605243404275*cos(q1L))/81129638414606681695789005144064 + (50055177836018480443110068268825*sin(q1L))/81129638414606681695789005144064 - 46293577452674263141823442369649/664613997892457936451903530140172288))/9007199254740992 + sin(q3L)*((55491554575214198102159220722265*sin(q2L))/162259276829213363391578010288128 + cos(q2L)*((5557241208790345*cos(q1L))/9007199254740992 - (6384186990310915*sin(q1L))/9007199254740992) + (7514214926474921*sin(q2L)*((6384186990310915*cos(q1L))/9007199254740992 + (5557241208790345*sin(q1L))/9007199254740992))/36893488147419103232)))/36893488147419103232 + ((7514214926474921*cos(q4L))/36893488147419103232 + (4503599440548691*sin(q4L))/4503599627370496)*((7514214926474921*sin(q3L)*((55491554575214198102159220722265*cos(q2L))/162259276829213363391578010288128 + (7514214926474921*cos(q2L)*((6384186990310915*cos(q1L))/9007199254740992 + (5557241208790345*sin(q1L))/9007199254740992))/36893488147419103232 - sin(q2L)*((5557241208790345*cos(q1L))/9007199254740992 - (6384186990310915*sin(q1L))/9007199254740992)))/36893488147419103232 - cos(q3L)*((55491554575214198102159220722265*sin(q2L))/162259276829213363391578010288128 + cos(q2L)*((5557241208790345*cos(q1L))/9007199254740992 - (6384186990310915*sin(q1L))/9007199254740992) + (7514214926474921*sin(q2L)*((6384186990310915*cos(q1L))/9007199254740992 + (5557241208790345*sin(q1L))/9007199254740992))/36893488147419103232) + (9007199067919185*sin(q3L)*((57503643108550260546605243404275*cos(q1L))/81129638414606681695789005144064 + (50055177836018480443110068268825*sin(q1L))/81129638414606681695789005144064 - 46293577452674263141823442369649/664613997892457936451903530140172288))/9007199254740992) - ((9007199067919185*cos(q4L))/9007199254740992 - (234819211581865*sin(q4L))/1152921504606846976)*((432094733372955093709245836907320566011451687275*cos(q1L))/2993155353253689176481146537402947624255349848014848 - (499823478647255911063139966257565597426350154025*cos(q2L))/1461501637330902918203684832716283019655932542976 + (376125364442766701270516501597006072214248637825*sin(q1L))/2993155353253689176481146537402947624255349848014848 - (67682029681889335677290557259385*cos(q2L)*((6384186990310915*cos(q1L))/9007199254740992 + (5557241208790345*sin(q1L))/9007199254740992))/332306998946228968225951765070086144 + (9007199067919185*sin(q2L)*((5557241208790345*cos(q1L))/9007199254740992 - (6384186990310915*sin(q1L))/9007199254740992))/9007199254740992 - 347859890694807798813742879236295256254610072729/24519928653854221733733552434404946937899825954937634816))))/9007199254740992000 + (48638874966763599*cos(q6L)*((5088386011442761075065519660541353066264654349799817218581453639893512373673125*cos(q1L))/4171849679533027504677776769862406473833407270227837441302815640277772901915313574263597826048 - (5885965739703093437427321469496047919878007806270640859921052774160471913354375*cos(q2L))/2037035976334486086268445688409378161051468393665936250636140449354381299763336706183397376 + (4429285744909692948152137219338012410016074630558523348687384033659145792819375*sin(q1L))/4171849679533027504677776769862406473833407270227837441302815640277772901915313574263597826048 + (67682029681889335677290557259385*cos(q4L)*((7514214926474921*cos(q3L)*((55491554575214198102159220722265*cos(q2L))/162259276829213363391578010288128 + (7514214926474921*cos(q2L)*((6384186990310915*cos(q1L))/9007199254740992 + (5557241208790345*sin(q1L))/9007199254740992))/36893488147419103232 - sin(q2L)*((5557241208790345*cos(q1L))/9007199254740992 - (6384186990310915*sin(q1L))/9007199254740992)))/36893488147419103232 + (9007199067919185*cos(q3L)*((57503643108550260546605243404275*cos(q1L))/81129638414606681695789005144064 + (50055177836018480443110068268825*sin(q1L))/81129638414606681695789005144064 - 46293577452674263141823442369649/664613997892457936451903530140172288))/9007199254740992 + sin(q3L)*((55491554575214198102159220722265*sin(q2L))/162259276829213363391578010288128 + cos(q2L)*((5557241208790345*cos(q1L))/9007199254740992 - (6384186990310915*sin(q1L))/9007199254740992) + (7514214926474921*sin(q2L)*((6384186990310915*cos(q1L))/9007199254740992 + (5557241208790345*sin(q1L))/9007199254740992))/36893488147419103232)))/332306998946228968225951765070086144 - (797029601289130257223357069404502671534492977261568326111352375*cos(q2L)*((6384186990310915*cos(q1L))/9007199254740992 + (5557241208790345*sin(q1L))/9007199254740992))/463168356949264781694283940034751631413079938662562256157830336031652518559744 + (106069577339469832923929692356850887620017617375*sin(q2L)*((5557241208790345*cos(q1L))/9007199254740992 - (6384186990310915*sin(q1L))/9007199254740992))/12554203470773361527671578846415332832204710888928069025792 + (9007199067919185*((4503599440548691*cos(q4L))/4503599627370496 - (7514214926474921*sin(q4L))/36893488147419103232)*((7514214926474921*sin(q3L)*((55491554575214198102159220722265*cos(q2L))/162259276829213363391578010288128 + (7514214926474921*cos(q2L)*((6384186990310915*cos(q1L))/9007199254740992 + (5557241208790345*sin(q1L))/9007199254740992))/36893488147419103232 - sin(q2L)*((5557241208790345*cos(q1L))/9007199254740992 - (6384186990310915*sin(q1L))/9007199254740992)))/36893488147419103232 - cos(q3L)*((55491554575214198102159220722265*sin(q2L))/162259276829213363391578010288128 + cos(q2L)*((5557241208790345*cos(q1L))/9007199254740992 - (6384186990310915*sin(q1L))/9007199254740992) + (7514214926474921*sin(q2L)*((6384186990310915*cos(q1L))/9007199254740992 + (5557241208790345*sin(q1L))/9007199254740992))/36893488147419103232) + (9007199067919185*sin(q3L)*((57503643108550260546605243404275*cos(q1L))/81129638414606681695789005144064 + (50055177836018480443110068268825*sin(q1L))/81129638414606681695789005144064 - 46293577452674263141823442369649/664613997892457936451903530140172288))/9007199254740992))/9007199254740992 - (508577317689771495245073589786522929324694383585*cos(q3L)*((55491554575214198102159220722265*cos(q2L))/162259276829213363391578010288128 + (7514214926474921*cos(q2L)*((6384186990310915*cos(q1L))/9007199254740992 + (5557241208790345*sin(q1L))/9007199254740992))/36893488147419103232 - sin(q2L)*((5557241208790345*cos(q1L))/9007199254740992 - (6384186990310915*sin(q1L))/9007199254740992)))/12259964326927110866866776217202473468949912977468817408 - (1764482024691522628700660907665*cos(q3L)*((55491554575214198102159220722265*sin(q2L))/162259276829213363391578010288128 + cos(q2L)*((5557241208790345*cos(q1L))/9007199254740992 - (6384186990310915*sin(q1L))/9007199254740992) + (7514214926474921*sin(q2L)*((6384186990310915*cos(q1L))/9007199254740992 + (5557241208790345*sin(q1L))/9007199254740992))/36893488147419103232))/42535295865117307932921825928971026432 + (13258697167433729449897784796786197386719169465*sin(q3L)*((55491554575214198102159220722265*cos(q2L))/162259276829213363391578010288128 + (7514214926474921*cos(q2L)*((6384186990310915*cos(q1L))/9007199254740992 + (5557241208790345*sin(q1L))/9007199254740992))/36893488147419103232 - sin(q2L)*((5557241208790345*cos(q1L))/9007199254740992 - (6384186990310915*sin(q1L))/9007199254740992)))/1569275433846670190958947355801916604025588861116008628224 - (609625514665592237562888769449172969868262801225*cos(q3L)*((57503643108550260546605243404275*cos(q1L))/81129638414606681695789005144064 + (50055177836018480443110068268825*sin(q1L))/81129638414606681695789005144064 - 46293577452674263141823442369649/664613997892457936451903530140172288))/2993155353253689176481146537402947624255349848014848 - (67682029681889335677290557259385*sin(q3L)*((55491554575214198102159220722265*sin(q2L))/162259276829213363391578010288128 + cos(q2L)*((5557241208790345*cos(q1L))/9007199254740992 - (6384186990310915*sin(q1L))/9007199254740992) + (7514214926474921*sin(q2L)*((6384186990310915*cos(q1L))/9007199254740992 + (5557241208790345*sin(q1L))/9007199254740992))/36893488147419103232))/332306998946228968225951765070086144 + (15893040848161638993908057577265778144967053025*sin(q3L)*((57503643108550260546605243404275*cos(q1L))/81129638414606681695789005144064 + (50055177836018480443110068268825*sin(q1L))/81129638414606681695789005144064 - 46293577452674263141823442369649/664613997892457936451903530140172288))/383123885216472214589586756787577295904684780545900544 + (9007199067919185*((234819211581865*cos(q4L))/1152921504606846976 + (9007199067919185*sin(q4L))/9007199254740992)*((432094733372955093709245836907320566011451687275*cos(q1L))/2993155353253689176481146537402947624255349848014848 - (499823478647255911063139966257565597426350154025*cos(q2L))/1461501637330902918203684832716283019655932542976 + (376125364442766701270516501597006072214248637825*sin(q1L))/2993155353253689176481146537402947624255349848014848 - (67682029681889335677290557259385*cos(q2L)*((6384186990310915*cos(q1L))/9007199254740992 + (5557241208790345*sin(q1L))/9007199254740992))/332306998946228968225951765070086144 + (9007199067919185*sin(q2L)*((5557241208790345*cos(q1L))/9007199254740992 - (6384186990310915*sin(q1L))/9007199254740992))/9007199254740992 - 347859890694807798813742879236295256254610072729/24519928653854221733733552434404946937899825954937634816))/9007199254740992 - 4096429012074266193201497846399339816506783348782596510723336809893932570711575/34175792574734561318320347298712833833643272357706444319152665725155515612490248800367393390985216))/1801439850948198400 + (27*sin(q6L)*((9007199067919185*sin(q5L)*((783310804561232573774573497517025067305577458842146606386579375*cos(q2L))/55213970774324510299478046898216203619608871777363092441300193790394368 - (677168015718420743488926864722853474412798830140650728756148125*cos(q1L))/113078212145816597093331040047546785012958969400039613319782796882727665664 - (589454226189876320500100500762517606499114263738369612804244375*sin(q1L))/113078212145816597093331040047546785012958969400039613319782796882727665664 + (106069577339469832923929692356850887620017617375*cos(q2L)*((6384186990310915*cos(q1L))/9007199254740992 + (5557241208790345*sin(q1L))/9007199254740992))/12554203470773361527671578846415332832204710888928069025792 - (14115856197532180673579726082375*sin(q2L)*((5557241208790345*cos(q1L))/9007199254740992 - (6384186990310915*sin(q1L))/9007199254740992))/340282366920938463463374607431768211456 + (67682029681889335677290557259385*cos(q3L)*((55491554575214198102159220722265*cos(q2L))/162259276829213363391578010288128 + (7514214926474921*cos(q2L)*((6384186990310915*cos(q1L))/9007199254740992 + (5557241208790345*sin(q1L))/9007199254740992))/36893488147419103232 - sin(q2L)*((5557241208790345*cos(q1L))/9007199254740992 - (6384186990310915*sin(q1L))/9007199254740992)))/332306998946228968225951765070086144 + (234819211581865*cos(q3L)*((55491554575214198102159220722265*sin(q2L))/162259276829213363391578010288128 + cos(q2L)*((5557241208790345*cos(q1L))/9007199254740992 - (6384186990310915*sin(q1L))/9007199254740992) + (7514214926474921*sin(q2L)*((6384186990310915*cos(q1L))/9007199254740992 + (5557241208790345*sin(q1L))/9007199254740992))/36893488147419103232))/1152921504606846976 - (1764482024691522628700660907665*sin(q3L)*((55491554575214198102159220722265*cos(q2L))/162259276829213363391578010288128 + (7514214926474921*cos(q2L)*((6384186990310915*cos(q1L))/9007199254740992 + (5557241208790345*sin(q1L))/9007199254740992))/36893488147419103232 - sin(q2L)*((5557241208790345*cos(q1L))/9007199254740992 - (6384186990310915*sin(q1L))/9007199254740992)))/42535295865117307932921825928971026432 + (81129635049124235038645691064225*cos(q3L)*((57503643108550260546605243404275*cos(q1L))/81129638414606681695789005144064 + (50055177836018480443110068268825*sin(q1L))/81129638414606681695789005144064 - 46293577452674263141823442369649/664613997892457936451903530140172288))/81129638414606681695789005144064 + (9007199067919185*sin(q3L)*((55491554575214198102159220722265*sin(q2L))/162259276829213363391578010288128 + cos(q2L)*((5557241208790345*cos(q1L))/9007199254740992 - (6384186990310915*sin(q1L))/9007199254740992) + (7514214926474921*sin(q2L)*((6384186990310915*cos(q1L))/9007199254740992 + (5557241208790345*sin(q1L))/9007199254740992))/36893488147419103232))/9007199254740992 - (2115063383689692319117831580025*sin(q3L)*((57503643108550260546605243404275*cos(q1L))/81129638414606681695789005144064 + (50055177836018480443110068268825*sin(q1L))/81129638414606681695789005144064 - 46293577452674263141823442369649/664613997892457936451903530140172288))/10384593717069655257060992658440192 + 545157285512458543963749743061519108960107968042455893206992575/926336713898529563388567880069503262826159877325124512315660672063305037119488))/9007199254740992 + (7514214926474921*sin(q5L)*((7514214926474921*cos(q4L)*((7514214926474921*cos(q3L)*((55491554575214198102159220722265*cos(q2L))/162259276829213363391578010288128 + (7514214926474921*cos(q2L)*((6384186990310915*cos(q1L))/9007199254740992 + (5557241208790345*sin(q1L))/9007199254740992))/36893488147419103232 - sin(q2L)*((5557241208790345*cos(q1L))/9007199254740992 - (6384186990310915*sin(q1L))/9007199254740992)))/36893488147419103232 + (9007199067919185*cos(q3L)*((57503643108550260546605243404275*cos(q1L))/81129638414606681695789005144064 + (50055177836018480443110068268825*sin(q1L))/81129638414606681695789005144064 - 46293577452674263141823442369649/664613997892457936451903530140172288))/9007199254740992 + sin(q3L)*((55491554575214198102159220722265*sin(q2L))/162259276829213363391578010288128 + cos(q2L)*((5557241208790345*cos(q1L))/9007199254740992 - (6384186990310915*sin(q1L))/9007199254740992) + (7514214926474921*sin(q2L)*((6384186990310915*cos(q1L))/9007199254740992 + (5557241208790345*sin(q1L))/9007199254740992))/36893488147419103232)))/36893488147419103232 + ((4503599440548691*cos(q4L))/4503599627370496 - (7514214926474921*sin(q4L))/36893488147419103232)*((7514214926474921*sin(q3L)*((55491554575214198102159220722265*cos(q2L))/162259276829213363391578010288128 + (7514214926474921*cos(q2L)*((6384186990310915*cos(q1L))/9007199254740992 + (5557241208790345*sin(q1L))/9007199254740992))/36893488147419103232 - sin(q2L)*((5557241208790345*cos(q1L))/9007199254740992 - (6384186990310915*sin(q1L))/9007199254740992)))/36893488147419103232 - cos(q3L)*((55491554575214198102159220722265*sin(q2L))/162259276829213363391578010288128 + cos(q2L)*((5557241208790345*cos(q1L))/9007199254740992 - (6384186990310915*sin(q1L))/9007199254740992) + (7514214926474921*sin(q2L)*((6384186990310915*cos(q1L))/9007199254740992 + (5557241208790345*sin(q1L))/9007199254740992))/36893488147419103232) + (9007199067919185*sin(q3L)*((57503643108550260546605243404275*cos(q1L))/81129638414606681695789005144064 + (50055177836018480443110068268825*sin(q1L))/81129638414606681695789005144064 - 46293577452674263141823442369649/664613997892457936451903530140172288))/9007199254740992) + ((234819211581865*cos(q4L))/1152921504606846976 + (9007199067919185*sin(q4L))/9007199254740992)*((432094733372955093709245836907320566011451687275*cos(q1L))/2993155353253689176481146537402947624255349848014848 - (499823478647255911063139966257565597426350154025*cos(q2L))/1461501637330902918203684832716283019655932542976 + (376125364442766701270516501597006072214248637825*sin(q1L))/2993155353253689176481146537402947624255349848014848 - (67682029681889335677290557259385*cos(q2L)*((6384186990310915*cos(q1L))/9007199254740992 + (5557241208790345*sin(q1L))/9007199254740992))/332306998946228968225951765070086144 + (9007199067919185*sin(q2L)*((5557241208790345*cos(q1L))/9007199254740992 - (6384186990310915*sin(q1L))/9007199254740992))/9007199254740992 - 347859890694807798813742879236295256254610072729/24519928653854221733733552434404946937899825954937634816)))/36893488147419103232 - cos(q5L)*((7514214926474921*sin(q4L)*((7514214926474921*cos(q3L)*((55491554575214198102159220722265*cos(q2L))/162259276829213363391578010288128 + (7514214926474921*cos(q2L)*((6384186990310915*cos(q1L))/9007199254740992 + (5557241208790345*sin(q1L))/9007199254740992))/36893488147419103232 - sin(q2L)*((5557241208790345*cos(q1L))/9007199254740992 - (6384186990310915*sin(q1L))/9007199254740992)))/36893488147419103232 + (9007199067919185*cos(q3L)*((57503643108550260546605243404275*cos(q1L))/81129638414606681695789005144064 + (50055177836018480443110068268825*sin(q1L))/81129638414606681695789005144064 - 46293577452674263141823442369649/664613997892457936451903530140172288))/9007199254740992 + sin(q3L)*((55491554575214198102159220722265*sin(q2L))/162259276829213363391578010288128 + cos(q2L)*((5557241208790345*cos(q1L))/9007199254740992 - (6384186990310915*sin(q1L))/9007199254740992) + (7514214926474921*sin(q2L)*((6384186990310915*cos(q1L))/9007199254740992 + (5557241208790345*sin(q1L))/9007199254740992))/36893488147419103232)))/36893488147419103232 + ((7514214926474921*cos(q4L))/36893488147419103232 + (4503599440548691*sin(q4L))/4503599627370496)*((7514214926474921*sin(q3L)*((55491554575214198102159220722265*cos(q2L))/162259276829213363391578010288128 + (7514214926474921*cos(q2L)*((6384186990310915*cos(q1L))/9007199254740992 + (5557241208790345*sin(q1L))/9007199254740992))/36893488147419103232 - sin(q2L)*((5557241208790345*cos(q1L))/9007199254740992 - (6384186990310915*sin(q1L))/9007199254740992)))/36893488147419103232 - cos(q3L)*((55491554575214198102159220722265*sin(q2L))/162259276829213363391578010288128 + cos(q2L)*((5557241208790345*cos(q1L))/9007199254740992 - (6384186990310915*sin(q1L))/9007199254740992) + (7514214926474921*sin(q2L)*((6384186990310915*cos(q1L))/9007199254740992 + (5557241208790345*sin(q1L))/9007199254740992))/36893488147419103232) + (9007199067919185*sin(q3L)*((57503643108550260546605243404275*cos(q1L))/81129638414606681695789005144064 + (50055177836018480443110068268825*sin(q1L))/81129638414606681695789005144064 - 46293577452674263141823442369649/664613997892457936451903530140172288))/9007199254740992) - ((9007199067919185*cos(q4L))/9007199254740992 - (234819211581865*sin(q4L))/1152921504606846976)*((432094733372955093709245836907320566011451687275*cos(q1L))/2993155353253689176481146537402947624255349848014848 - (499823478647255911063139966257565597426350154025*cos(q2L))/1461501637330902918203684832716283019655932542976 + (376125364442766701270516501597006072214248637825*sin(q1L))/2993155353253689176481146537402947624255349848014848 - (67682029681889335677290557259385*cos(q2L)*((6384186990310915*cos(q1L))/9007199254740992 + (5557241208790345*sin(q1L))/9007199254740992))/332306998946228968225951765070086144 + (9007199067919185*sin(q2L)*((5557241208790345*cos(q1L))/9007199254740992 - (6384186990310915*sin(q1L))/9007199254740992))/9007199254740992 - 347859890694807798813742879236295256254610072729/24519928653854221733733552434404946937899825954937634816))))/1000 - (584133382113593486367040631332731*sin(q6L)*((5088386011442761075065519660541353066264654349799817218581453639893512373673125*cos(q1L))/4171849679533027504677776769862406473833407270227837441302815640277772901915313574263597826048 - (5885965739703093437427321469496047919878007806270640859921052774160471913354375*cos(q2L))/2037035976334486086268445688409378161051468393665936250636140449354381299763336706183397376 + (4429285744909692948152137219338012410016074630558523348687384033659145792819375*sin(q1L))/4171849679533027504677776769862406473833407270227837441302815640277772901915313574263597826048 + (67682029681889335677290557259385*cos(q4L)*((7514214926474921*cos(q3L)*((55491554575214198102159220722265*cos(q2L))/162259276829213363391578010288128 + (7514214926474921*cos(q2L)*((6384186990310915*cos(q1L))/9007199254740992 + (5557241208790345*sin(q1L))/9007199254740992))/36893488147419103232 - sin(q2L)*((5557241208790345*cos(q1L))/9007199254740992 - (6384186990310915*sin(q1L))/9007199254740992)))/36893488147419103232 + (9007199067919185*cos(q3L)*((57503643108550260546605243404275*cos(q1L))/81129638414606681695789005144064 + (50055177836018480443110068268825*sin(q1L))/81129638414606681695789005144064 - 46293577452674263141823442369649/664613997892457936451903530140172288))/9007199254740992 + sin(q3L)*((55491554575214198102159220722265*sin(q2L))/162259276829213363391578010288128 + cos(q2L)*((5557241208790345*cos(q1L))/9007199254740992 - (6384186990310915*sin(q1L))/9007199254740992) + (7514214926474921*sin(q2L)*((6384186990310915*cos(q1L))/9007199254740992 + (5557241208790345*sin(q1L))/9007199254740992))/36893488147419103232)))/332306998946228968225951765070086144 - (797029601289130257223357069404502671534492977261568326111352375*cos(q2L)*((6384186990310915*cos(q1L))/9007199254740992 + (5557241208790345*sin(q1L))/9007199254740992))/463168356949264781694283940034751631413079938662562256157830336031652518559744 + (106069577339469832923929692356850887620017617375*sin(q2L)*((5557241208790345*cos(q1L))/9007199254740992 - (6384186990310915*sin(q1L))/9007199254740992))/12554203470773361527671578846415332832204710888928069025792 + (9007199067919185*((4503599440548691*cos(q4L))/4503599627370496 - (7514214926474921*sin(q4L))/36893488147419103232)*((7514214926474921*sin(q3L)*((55491554575214198102159220722265*cos(q2L))/162259276829213363391578010288128 + (7514214926474921*cos(q2L)*((6384186990310915*cos(q1L))/9007199254740992 + (5557241208790345*sin(q1L))/9007199254740992))/36893488147419103232 - sin(q2L)*((5557241208790345*cos(q1L))/9007199254740992 - (6384186990310915*sin(q1L))/9007199254740992)))/36893488147419103232 - cos(q3L)*((55491554575214198102159220722265*sin(q2L))/162259276829213363391578010288128 + cos(q2L)*((5557241208790345*cos(q1L))/9007199254740992 - (6384186990310915*sin(q1L))/9007199254740992) + (7514214926474921*sin(q2L)*((6384186990310915*cos(q1L))/9007199254740992 + (5557241208790345*sin(q1L))/9007199254740992))/36893488147419103232) + (9007199067919185*sin(q3L)*((57503643108550260546605243404275*cos(q1L))/81129638414606681695789005144064 + (50055177836018480443110068268825*sin(q1L))/81129638414606681695789005144064 - 46293577452674263141823442369649/664613997892457936451903530140172288))/9007199254740992))/9007199254740992 - (508577317689771495245073589786522929324694383585*cos(q3L)*((55491554575214198102159220722265*cos(q2L))/162259276829213363391578010288128 + (7514214926474921*cos(q2L)*((6384186990310915*cos(q1L))/9007199254740992 + (5557241208790345*sin(q1L))/9007199254740992))/36893488147419103232 - sin(q2L)*((5557241208790345*cos(q1L))/9007199254740992 - (6384186990310915*sin(q1L))/9007199254740992)))/12259964326927110866866776217202473468949912977468817408 - (1764482024691522628700660907665*cos(q3L)*((55491554575214198102159220722265*sin(q2L))/162259276829213363391578010288128 + cos(q2L)*((5557241208790345*cos(q1L))/9007199254740992 - (6384186990310915*sin(q1L))/9007199254740992) + (7514214926474921*sin(q2L)*((6384186990310915*cos(q1L))/9007199254740992 + (5557241208790345*sin(q1L))/9007199254740992))/36893488147419103232))/42535295865117307932921825928971026432 + (13258697167433729449897784796786197386719169465*sin(q3L)*((55491554575214198102159220722265*cos(q2L))/162259276829213363391578010288128 + (7514214926474921*cos(q2L)*((6384186990310915*cos(q1L))/9007199254740992 + (5557241208790345*sin(q1L))/9007199254740992))/36893488147419103232 - sin(q2L)*((5557241208790345*cos(q1L))/9007199254740992 - (6384186990310915*sin(q1L))/9007199254740992)))/1569275433846670190958947355801916604025588861116008628224 - (609625514665592237562888769449172969868262801225*cos(q3L)*((57503643108550260546605243404275*cos(q1L))/81129638414606681695789005144064 + (50055177836018480443110068268825*sin(q1L))/81129638414606681695789005144064 - 46293577452674263141823442369649/664613997892457936451903530140172288))/2993155353253689176481146537402947624255349848014848 - (67682029681889335677290557259385*sin(q3L)*((55491554575214198102159220722265*sin(q2L))/162259276829213363391578010288128 + cos(q2L)*((5557241208790345*cos(q1L))/9007199254740992 - (6384186990310915*sin(q1L))/9007199254740992) + (7514214926474921*sin(q2L)*((6384186990310915*cos(q1L))/9007199254740992 + (5557241208790345*sin(q1L))/9007199254740992))/36893488147419103232))/332306998946228968225951765070086144 + (15893040848161638993908057577265778144967053025*sin(q3L)*((57503643108550260546605243404275*cos(q1L))/81129638414606681695789005144064 + (50055177836018480443110068268825*sin(q1L))/81129638414606681695789005144064 - 46293577452674263141823442369649/664613997892457936451903530140172288))/383123885216472214589586756787577295904684780545900544 + (9007199067919185*((234819211581865*cos(q4L))/1152921504606846976 + (9007199067919185*sin(q4L))/9007199254740992)*((432094733372955093709245836907320566011451687275*cos(q1L))/2993155353253689176481146537402947624255349848014848 - (499823478647255911063139966257565597426350154025*cos(q2L))/1461501637330902918203684832716283019655932542976 + (376125364442766701270516501597006072214248637825*sin(q1L))/2993155353253689176481146537402947624255349848014848 - (67682029681889335677290557259385*cos(q2L)*((6384186990310915*cos(q1L))/9007199254740992 + (5557241208790345*sin(q1L))/9007199254740992))/332306998946228968225951765070086144 + (9007199067919185*sin(q2L)*((5557241208790345*cos(q1L))/9007199254740992 - (6384186990310915*sin(q1L))/9007199254740992))/9007199254740992 - 347859890694807798813742879236295256254610072729/24519928653854221733733552434404946937899825954937634816))/9007199254740992 - 4096429012074266193201497846399339816506783348782596510723336809893932570711575/34175792574734561318320347298712833833643272357706444319152665725155515612490248800367393390985216))/16225927682921336339157801028812800, 0; (593933483172578389632813415592295832530354254928157399102928396179289049509180830725931534345974379279786096209254972773983973140135897*cos(q1L))/28392137667797144162082961245625177123189115651848361729745710905493722191929606379929337918506389279717286000244772575528695376117760000 - (461103588256600777298885336820449355216197832651752567100077883927180554390938377031662943654755250981573943235862396074774396544535817*sin(q1L))/28392137667797144162082961245625177123189115651848361729745710905493722191929606379929337918506389279717286000244772575528695376117760000 + (170695144106365826517608855445768431563113584343*cos(q5L)*((516845254133432670685844229576986303733782399690601453662320875*cos(q1L))/113078212145816597093331040047546785012958969400039613319782796882727665664 + (666467732349846997487583938718911583194406904318712922873589125*sin(q1L))/113078212145816597093331040047546785012958969400039613319782796882727665664 - (9007199067919185*sin(q3L)*(cos(q2L)*((6283307137322267*cos(q1L))/9007199254740992 - (4872700232219253*sin(q1L))/9007199254740992) + (7514214926474921*sin(q2L)*((4872700232219253*cos(q1L))/9007199254740992 + (6283307137322267*sin(q1L))/9007199254740992))/36893488147419103232))/9007199254740992 + (1764482024691522628700660907665*sin(q3L)*((7514214926474921*cos(q2L)*((4872700232219253*cos(q1L))/9007199254740992 + (6283307137322267*sin(q1L))/9007199254740992))/36893488147419103232 - sin(q2L)*((6283307137322267*cos(q1L))/9007199254740992 - (4872700232219253*sin(q1L))/9007199254740992)))/42535295865117307932921825928971026432 - (106069577339469832923929692356850887620017617375*cos(q2L)*((4872700232219253*cos(q1L))/9007199254740992 + (6283307137322267*sin(q1L))/9007199254740992))/12554203470773361527671578846415332832204710888928069025792 + (14115856197532180673579726082375*sin(q2L)*((6283307137322267*cos(q1L))/9007199254740992 - (4872700232219253*sin(q1L))/9007199254740992))/340282366920938463463374607431768211456 - (81129635049124235038645691064225*cos(q3L)*((43889380989894851923989405068805*cos(q1L))/81129638414606681695789005144064 + (56594998190739085871744456992395*sin(q1L))/81129638414606681695789005144064))/81129638414606681695789005144064 + (2115063383689692319117831580025*sin(q3L)*((43889380989894851923989405068805*cos(q1L))/81129638414606681695789005144064 + (56594998190739085871744456992395*sin(q1L))/81129638414606681695789005144064))/10384593717069655257060992658440192 - (234819211581865*cos(q3L)*(cos(q2L)*((6283307137322267*cos(q1L))/9007199254740992 - (4872700232219253*sin(q1L))/9007199254740992) + (7514214926474921*sin(q2L)*((4872700232219253*cos(q1L))/9007199254740992 + (6283307137322267*sin(q1L))/9007199254740992))/36893488147419103232))/1152921504606846976 - (67682029681889335677290557259385*cos(q3L)*((7514214926474921*cos(q2L)*((4872700232219253*cos(q1L))/9007199254740992 + (6283307137322267*sin(q1L))/9007199254740992))/36893488147419103232 - sin(q2L)*((6283307137322267*cos(q1L))/9007199254740992 - (4872700232219253*sin(q1L))/9007199254740992)))/332306998946228968225951765070086144))/119726214130147567059245861496117904970213993920593920 - (46241644459901303158631016767207157814229090534989303509431886332469146043*sin(q3L)*(cos(q2L)*((6283307137322267*cos(q1L))/9007199254740992 - (4872700232219253*sin(q1L))/9007199254740992) + (7514214926474921*sin(q2L)*((4872700232219253*cos(q1L))/9007199254740992 + (6283307137322267*sin(q1L))/9007199254740992))/36893488147419103232))/2261564242916331941866620800950935700259179388000792266395655937654553313280000 + (455490404115240510935077772268745492204390157443214084883134054419271951750419293234291596923751*sin(q3L)*((7514214926474921*cos(q2L)*((4872700232219253*cos(q1L))/9007199254740992 + (6283307137322267*sin(q1L))/9007199254740992))/36893488147419103232 - sin(q2L)*((6283307137322267*cos(q1L))/9007199254740992 - (4872700232219253*sin(q1L))/9007199254740992)))/53399675898022752059875542654238802865067613058916319248676040195555493144516013750574052173414400000 - (48638874966763599*sin(q5L)*((516845254133432670685844229576986303733782399690601453662320875*cos(q1L))/113078212145816597093331040047546785012958969400039613319782796882727665664 + (666467732349846997487583938718911583194406904318712922873589125*sin(q1L))/113078212145816597093331040047546785012958969400039613319782796882727665664 - (9007199067919185*sin(q3L)*(cos(q2L)*((6283307137322267*cos(q1L))/9007199254740992 - (4872700232219253*sin(q1L))/9007199254740992) + (7514214926474921*sin(q2L)*((4872700232219253*cos(q1L))/9007199254740992 + (6283307137322267*sin(q1L))/9007199254740992))/36893488147419103232))/9007199254740992 + (1764482024691522628700660907665*sin(q3L)*((7514214926474921*cos(q2L)*((4872700232219253*cos(q1L))/9007199254740992 + (6283307137322267*sin(q1L))/9007199254740992))/36893488147419103232 - sin(q2L)*((6283307137322267*cos(q1L))/9007199254740992 - (4872700232219253*sin(q1L))/9007199254740992)))/42535295865117307932921825928971026432 - (106069577339469832923929692356850887620017617375*cos(q2L)*((4872700232219253*cos(q1L))/9007199254740992 + (6283307137322267*sin(q1L))/9007199254740992))/12554203470773361527671578846415332832204710888928069025792 + (14115856197532180673579726082375*sin(q2L)*((6283307137322267*cos(q1L))/9007199254740992 - (4872700232219253*sin(q1L))/9007199254740992))/340282366920938463463374607431768211456 - (81129635049124235038645691064225*cos(q3L)*((43889380989894851923989405068805*cos(q1L))/81129638414606681695789005144064 + (56594998190739085871744456992395*sin(q1L))/81129638414606681695789005144064))/81129638414606681695789005144064 + (2115063383689692319117831580025*sin(q3L)*((43889380989894851923989405068805*cos(q1L))/81129638414606681695789005144064 + (56594998190739085871744456992395*sin(q1L))/81129638414606681695789005144064))/10384593717069655257060992658440192 - (234819211581865*cos(q3L)*(cos(q2L)*((6283307137322267*cos(q1L))/9007199254740992 - (4872700232219253*sin(q1L))/9007199254740992) + (7514214926474921*sin(q2L)*((4872700232219253*cos(q1L))/9007199254740992 + (6283307137322267*sin(q1L))/9007199254740992))/36893488147419103232))/1152921504606846976 - (67682029681889335677290557259385*cos(q3L)*((7514214926474921*cos(q2L)*((4872700232219253*cos(q1L))/9007199254740992 + (6283307137322267*sin(q1L))/9007199254740992))/36893488147419103232 - sin(q2L)*((6283307137322267*cos(q1L))/9007199254740992 - (4872700232219253*sin(q1L))/9007199254740992)))/332306998946228968225951765070086144))/1801439850948198400 + (584133382113593486367040631332731*cos(q6L)*((3883686323287163634621917344193152976968889150546766896070169015701143342275875*cos(q1L))/4171849679533027504677776769862406473833407270227837441302815640277772901915313574263597826048 + (5007981782437112884252809417893315588674027328151397427571757674310327570834125*sin(q1L))/4171849679533027504677776769862406473833407270227837441302815640277772901915313574263597826048 - (67682029681889335677290557259385*sin(q3L)*(cos(q2L)*((6283307137322267*cos(q1L))/9007199254740992 - (4872700232219253*sin(q1L))/9007199254740992) + (7514214926474921*sin(q2L)*((4872700232219253*cos(q1L))/9007199254740992 + (6283307137322267*sin(q1L))/9007199254740992))/36893488147419103232))/332306998946228968225951765070086144 + (13258697167433729449897784796786197386719169465*sin(q3L)*((7514214926474921*cos(q2L)*((4872700232219253*cos(q1L))/9007199254740992 + (6283307137322267*sin(q1L))/9007199254740992))/36893488147419103232 - sin(q2L)*((6283307137322267*cos(q1L))/9007199254740992 - (4872700232219253*sin(q1L))/9007199254740992)))/1569275433846670190958947355801916604025588861116008628224 + (9007199067919185*((234819211581865*cos(q4L))/1152921504606846976 + (9007199067919185*sin(q4L))/9007199254740992)*((329794241748012540206902858004467560228111939405*cos(q1L))/2993155353253689176481146537402947624255349848014848 + (425266980168672787164801917791314326747055225795*sin(q1L))/2993155353253689176481146537402947624255349848014848 - (67682029681889335677290557259385*cos(q2L)*((4872700232219253*cos(q1L))/9007199254740992 + (6283307137322267*sin(q1L))/9007199254740992))/332306998946228968225951765070086144 + (9007199067919185*sin(q2L)*((6283307137322267*cos(q1L))/9007199254740992 - (4872700232219253*sin(q1L))/9007199254740992))/9007199254740992))/9007199254740992 + (9007199067919185*((4503599440548691*cos(q4L))/4503599627370496 - (7514214926474921*sin(q4L))/36893488147419103232)*((7514214926474921*sin(q3L)*((7514214926474921*cos(q2L)*((4872700232219253*cos(q1L))/9007199254740992 + (6283307137322267*sin(q1L))/9007199254740992))/36893488147419103232 - sin(q2L)*((6283307137322267*cos(q1L))/9007199254740992 - (4872700232219253*sin(q1L))/9007199254740992)))/36893488147419103232 + (9007199067919185*sin(q3L)*((43889380989894851923989405068805*cos(q1L))/81129638414606681695789005144064 + (56594998190739085871744456992395*sin(q1L))/81129638414606681695789005144064))/9007199254740992 - cos(q3L)*(cos(q2L)*((6283307137322267*cos(q1L))/9007199254740992 - (4872700232219253*sin(q1L))/9007199254740992) + (7514214926474921*sin(q2L)*((4872700232219253*cos(q1L))/9007199254740992 + (6283307137322267*sin(q1L))/9007199254740992))/36893488147419103232)))/9007199254740992 - (797029601289130257223357069404502671534492977261568326111352375*cos(q2L)*((4872700232219253*cos(q1L))/9007199254740992 + (6283307137322267*sin(q1L))/9007199254740992))/463168356949264781694283940034751631413079938662562256157830336031652518559744 + (106069577339469832923929692356850887620017617375*sin(q2L)*((6283307137322267*cos(q1L))/9007199254740992 - (4872700232219253*sin(q1L))/9007199254740992))/12554203470773361527671578846415332832204710888928069025792 - (609625514665592237562888769449172969868262801225*cos(q3L)*((43889380989894851923989405068805*cos(q1L))/81129638414606681695789005144064 + (56594998190739085871744456992395*sin(q1L))/81129638414606681695789005144064))/2993155353253689176481146537402947624255349848014848 + (67682029681889335677290557259385*cos(q4L)*(sin(q3L)*(cos(q2L)*((6283307137322267*cos(q1L))/9007199254740992 - (4872700232219253*sin(q1L))/9007199254740992) + (7514214926474921*sin(q2L)*((4872700232219253*cos(q1L))/9007199254740992 + (6283307137322267*sin(q1L))/9007199254740992))/36893488147419103232) + (9007199067919185*cos(q3L)*((43889380989894851923989405068805*cos(q1L))/81129638414606681695789005144064 + (56594998190739085871744456992395*sin(q1L))/81129638414606681695789005144064))/9007199254740992 + (7514214926474921*cos(q3L)*((7514214926474921*cos(q2L)*((4872700232219253*cos(q1L))/9007199254740992 + (6283307137322267*sin(q1L))/9007199254740992))/36893488147419103232 - sin(q2L)*((6283307137322267*cos(q1L))/9007199254740992 - (4872700232219253*sin(q1L))/9007199254740992)))/36893488147419103232))/332306998946228968225951765070086144 + (15893040848161638993908057577265778144967053025*sin(q3L)*((43889380989894851923989405068805*cos(q1L))/81129638414606681695789005144064 + (56594998190739085871744456992395*sin(q1L))/81129638414606681695789005144064))/383123885216472214589586756787577295904684780545900544 - (1764482024691522628700660907665*cos(q3L)*(cos(q2L)*((6283307137322267*cos(q1L))/9007199254740992 - (4872700232219253*sin(q1L))/9007199254740992) + (7514214926474921*sin(q2L)*((4872700232219253*cos(q1L))/9007199254740992 + (6283307137322267*sin(q1L))/9007199254740992))/36893488147419103232))/42535295865117307932921825928971026432 - (508577317689771495245073589786522929324694383585*cos(q3L)*((7514214926474921*cos(q2L)*((4872700232219253*cos(q1L))/9007199254740992 + (6283307137322267*sin(q1L))/9007199254740992))/36893488147419103232 - sin(q2L)*((6283307137322267*cos(q1L))/9007199254740992 - (4872700232219253*sin(q1L))/9007199254740992)))/12259964326927110866866776217202473468949912977468817408))/16225927682921336339157801028812800 - (81*((9007199067919185*cos(q4L))/9007199254740992 - (234819211581865*sin(q4L))/1152921504606846976)*((329794241748012540206902858004467560228111939405*cos(q1L))/2993155353253689176481146537402947624255349848014848 + (425266980168672787164801917791314326747055225795*sin(q1L))/2993155353253689176481146537402947624255349848014848 - (67682029681889335677290557259385*cos(q2L)*((4872700232219253*cos(q1L))/9007199254740992 + (6283307137322267*sin(q1L))/9007199254740992))/332306998946228968225951765070086144 + (9007199067919185*sin(q2L)*((6283307137322267*cos(q1L))/9007199254740992 - (4872700232219253*sin(q1L))/9007199254740992))/9007199254740992))/2000 + (81222263116692158804177042061221826384594597321566869716687*((234819211581865*cos(q4L))/1152921504606846976 + (9007199067919185*sin(q4L))/9007199254740992)*((329794241748012540206902858004467560228111939405*cos(q1L))/2993155353253689176481146537402947624255349848014848 + (425266980168672787164801917791314326747055225795*sin(q1L))/2993155353253689176481146537402947624255349848014848 - (67682029681889335677290557259385*cos(q2L)*((4872700232219253*cos(q1L))/9007199254740992 + (6283307137322267*sin(q1L))/9007199254740992))/332306998946228968225951765070086144 + (9007199067919185*sin(q2L)*((6283307137322267*cos(q1L))/9007199254740992 - (4872700232219253*sin(q1L))/9007199254740992))/9007199254740992))/306499108173177771671669405430061836723747824436720435200000 + (81222263116692158804177042061221826384594597321566869716687*((4503599440548691*cos(q4L))/4503599627370496 - (7514214926474921*sin(q4L))/36893488147419103232)*((7514214926474921*sin(q3L)*((7514214926474921*cos(q2L)*((4872700232219253*cos(q1L))/9007199254740992 + (6283307137322267*sin(q1L))/9007199254740992))/36893488147419103232 - sin(q2L)*((6283307137322267*cos(q1L))/9007199254740992 - (4872700232219253*sin(q1L))/9007199254740992)))/36893488147419103232 + (9007199067919185*sin(q3L)*((43889380989894851923989405068805*cos(q1L))/81129638414606681695789005144064 + (56594998190739085871744456992395*sin(q1L))/81129638414606681695789005144064))/9007199254740992 - cos(q3L)*(cos(q2L)*((6283307137322267*cos(q1L))/9007199254740992 - (4872700232219253*sin(q1L))/9007199254740992) + (7514214926474921*sin(q2L)*((4872700232219253*cos(q1L))/9007199254740992 + (6283307137322267*sin(q1L))/9007199254740992))/36893488147419103232)))/306499108173177771671669405430061836723747824436720435200000 + (81*((7514214926474921*cos(q4L))/36893488147419103232 + (4503599440548691*sin(q4L))/4503599627370496)*((7514214926474921*sin(q3L)*((7514214926474921*cos(q2L)*((4872700232219253*cos(q1L))/9007199254740992 + (6283307137322267*sin(q1L))/9007199254740992))/36893488147419103232 - sin(q2L)*((6283307137322267*cos(q1L))/9007199254740992 - (4872700232219253*sin(q1L))/9007199254740992)))/36893488147419103232 + (9007199067919185*sin(q3L)*((43889380989894851923989405068805*cos(q1L))/81129638414606681695789005144064 + (56594998190739085871744456992395*sin(q1L))/81129638414606681695789005144064))/9007199254740992 - cos(q3L)*(cos(q2L)*((6283307137322267*cos(q1L))/9007199254740992 - (4872700232219253*sin(q1L))/9007199254740992) + (7514214926474921*sin(q2L)*((4872700232219253*cos(q1L))/9007199254740992 + (6283307137322267*sin(q1L))/9007199254740992))/36893488147419103232)))/2000 + (48638874966763599*sin(q6L)*((3883686323287163634621917344193152976968889150546766896070169015701143342275875*cos(q1L))/4171849679533027504677776769862406473833407270227837441302815640277772901915313574263597826048 + (5007981782437112884252809417893315588674027328151397427571757674310327570834125*sin(q1L))/4171849679533027504677776769862406473833407270227837441302815640277772901915313574263597826048 - (67682029681889335677290557259385*sin(q3L)*(cos(q2L)*((6283307137322267*cos(q1L))/9007199254740992 - (4872700232219253*sin(q1L))/9007199254740992) + (7514214926474921*sin(q2L)*((4872700232219253*cos(q1L))/9007199254740992 + (6283307137322267*sin(q1L))/9007199254740992))/36893488147419103232))/332306998946228968225951765070086144 + (13258697167433729449897784796786197386719169465*sin(q3L)*((7514214926474921*cos(q2L)*((4872700232219253*cos(q1L))/9007199254740992 + (6283307137322267*sin(q1L))/9007199254740992))/36893488147419103232 - sin(q2L)*((6283307137322267*cos(q1L))/9007199254740992 - (4872700232219253*sin(q1L))/9007199254740992)))/1569275433846670190958947355801916604025588861116008628224 + (9007199067919185*((234819211581865*cos(q4L))/1152921504606846976 + (9007199067919185*sin(q4L))/9007199254740992)*((329794241748012540206902858004467560228111939405*cos(q1L))/2993155353253689176481146537402947624255349848014848 + (425266980168672787164801917791314326747055225795*sin(q1L))/2993155353253689176481146537402947624255349848014848 - (67682029681889335677290557259385*cos(q2L)*((4872700232219253*cos(q1L))/9007199254740992 + (6283307137322267*sin(q1L))/9007199254740992))/332306998946228968225951765070086144 + (9007199067919185*sin(q2L)*((6283307137322267*cos(q1L))/9007199254740992 - (4872700232219253*sin(q1L))/9007199254740992))/9007199254740992))/9007199254740992 + (9007199067919185*((4503599440548691*cos(q4L))/4503599627370496 - (7514214926474921*sin(q4L))/36893488147419103232)*((7514214926474921*sin(q3L)*((7514214926474921*cos(q2L)*((4872700232219253*cos(q1L))/9007199254740992 + (6283307137322267*sin(q1L))/9007199254740992))/36893488147419103232 - sin(q2L)*((6283307137322267*cos(q1L))/9007199254740992 - (4872700232219253*sin(q1L))/9007199254740992)))/36893488147419103232 + (9007199067919185*sin(q3L)*((43889380989894851923989405068805*cos(q1L))/81129638414606681695789005144064 + (56594998190739085871744456992395*sin(q1L))/81129638414606681695789005144064))/9007199254740992 - cos(q3L)*(cos(q2L)*((6283307137322267*cos(q1L))/9007199254740992 - (4872700232219253*sin(q1L))/9007199254740992) + (7514214926474921*sin(q2L)*((4872700232219253*cos(q1L))/9007199254740992 + (6283307137322267*sin(q1L))/9007199254740992))/36893488147419103232)))/9007199254740992 - (797029601289130257223357069404502671534492977261568326111352375*cos(q2L)*((4872700232219253*cos(q1L))/9007199254740992 + (6283307137322267*sin(q1L))/9007199254740992))/463168356949264781694283940034751631413079938662562256157830336031652518559744 + (106069577339469832923929692356850887620017617375*sin(q2L)*((6283307137322267*cos(q1L))/9007199254740992 - (4872700232219253*sin(q1L))/9007199254740992))/12554203470773361527671578846415332832204710888928069025792 - (609625514665592237562888769449172969868262801225*cos(q3L)*((43889380989894851923989405068805*cos(q1L))/81129638414606681695789005144064 + (56594998190739085871744456992395*sin(q1L))/81129638414606681695789005144064))/2993155353253689176481146537402947624255349848014848 + (67682029681889335677290557259385*cos(q4L)*(sin(q3L)*(cos(q2L)*((6283307137322267*cos(q1L))/9007199254740992 - (4872700232219253*sin(q1L))/9007199254740992) + (7514214926474921*sin(q2L)*((4872700232219253*cos(q1L))/9007199254740992 + (6283307137322267*sin(q1L))/9007199254740992))/36893488147419103232) + (9007199067919185*cos(q3L)*((43889380989894851923989405068805*cos(q1L))/81129638414606681695789005144064 + (56594998190739085871744456992395*sin(q1L))/81129638414606681695789005144064))/9007199254740992 + (7514214926474921*cos(q3L)*((7514214926474921*cos(q2L)*((4872700232219253*cos(q1L))/9007199254740992 + (6283307137322267*sin(q1L))/9007199254740992))/36893488147419103232 - sin(q2L)*((6283307137322267*cos(q1L))/9007199254740992 - (4872700232219253*sin(q1L))/9007199254740992)))/36893488147419103232))/332306998946228968225951765070086144 + (15893040848161638993908057577265778144967053025*sin(q3L)*((43889380989894851923989405068805*cos(q1L))/81129638414606681695789005144064 + (56594998190739085871744456992395*sin(q1L))/81129638414606681695789005144064))/383123885216472214589586756787577295904684780545900544 - (1764482024691522628700660907665*cos(q3L)*(cos(q2L)*((6283307137322267*cos(q1L))/9007199254740992 - (4872700232219253*sin(q1L))/9007199254740992) + (7514214926474921*sin(q2L)*((4872700232219253*cos(q1L))/9007199254740992 + (6283307137322267*sin(q1L))/9007199254740992))/36893488147419103232))/42535295865117307932921825928971026432 - (508577317689771495245073589786522929324694383585*cos(q3L)*((7514214926474921*cos(q2L)*((4872700232219253*cos(q1L))/9007199254740992 + (6283307137322267*sin(q1L))/9007199254740992))/36893488147419103232 - sin(q2L)*((6283307137322267*cos(q1L))/9007199254740992 - (4872700232219253*sin(q1L))/9007199254740992)))/12259964326927110866866776217202473468949912977468817408))/1801439850948198400 + (2436553109258773196144549622003023*cos(q6L)*((7514214926474921*cos(q5L)*(((234819211581865*cos(q4L))/1152921504606846976 + (9007199067919185*sin(q4L))/9007199254740992)*((329794241748012540206902858004467560228111939405*cos(q1L))/2993155353253689176481146537402947624255349848014848 + (425266980168672787164801917791314326747055225795*sin(q1L))/2993155353253689176481146537402947624255349848014848 - (67682029681889335677290557259385*cos(q2L)*((4872700232219253*cos(q1L))/9007199254740992 + (6283307137322267*sin(q1L))/9007199254740992))/332306998946228968225951765070086144 + (9007199067919185*sin(q2L)*((6283307137322267*cos(q1L))/9007199254740992 - (4872700232219253*sin(q1L))/9007199254740992))/9007199254740992) + ((4503599440548691*cos(q4L))/4503599627370496 - (7514214926474921*sin(q4L))/36893488147419103232)*((7514214926474921*sin(q3L)*((7514214926474921*cos(q2L)*((4872700232219253*cos(q1L))/9007199254740992 + (6283307137322267*sin(q1L))/9007199254740992))/36893488147419103232 - sin(q2L)*((6283307137322267*cos(q1L))/9007199254740992 - (4872700232219253*sin(q1L))/9007199254740992)))/36893488147419103232 + (9007199067919185*sin(q3L)*((43889380989894851923989405068805*cos(q1L))/81129638414606681695789005144064 + (56594998190739085871744456992395*sin(q1L))/81129638414606681695789005144064))/9007199254740992 - cos(q3L)*(cos(q2L)*((6283307137322267*cos(q1L))/9007199254740992 - (4872700232219253*sin(q1L))/9007199254740992) + (7514214926474921*sin(q2L)*((4872700232219253*cos(q1L))/9007199254740992 + (6283307137322267*sin(q1L))/9007199254740992))/36893488147419103232)) + (7514214926474921*cos(q4L)*(sin(q3L)*(cos(q2L)*((6283307137322267*cos(q1L))/9007199254740992 - (4872700232219253*sin(q1L))/9007199254740992) + (7514214926474921*sin(q2L)*((4872700232219253*cos(q1L))/9007199254740992 + (6283307137322267*sin(q1L))/9007199254740992))/36893488147419103232) + (9007199067919185*cos(q3L)*((43889380989894851923989405068805*cos(q1L))/81129638414606681695789005144064 + (56594998190739085871744456992395*sin(q1L))/81129638414606681695789005144064))/9007199254740992 + (7514214926474921*cos(q3L)*((7514214926474921*cos(q2L)*((4872700232219253*cos(q1L))/9007199254740992 + (6283307137322267*sin(q1L))/9007199254740992))/36893488147419103232 - sin(q2L)*((6283307137322267*cos(q1L))/9007199254740992 - (4872700232219253*sin(q1L))/9007199254740992)))/36893488147419103232))/36893488147419103232))/36893488147419103232 - (9007199067919185*cos(q5L)*((516845254133432670685844229576986303733782399690601453662320875*cos(q1L))/113078212145816597093331040047546785012958969400039613319782796882727665664 + (666467732349846997487583938718911583194406904318712922873589125*sin(q1L))/113078212145816597093331040047546785012958969400039613319782796882727665664 - (9007199067919185*sin(q3L)*(cos(q2L)*((6283307137322267*cos(q1L))/9007199254740992 - (4872700232219253*sin(q1L))/9007199254740992) + (7514214926474921*sin(q2L)*((4872700232219253*cos(q1L))/9007199254740992 + (6283307137322267*sin(q1L))/9007199254740992))/36893488147419103232))/9007199254740992 + (1764482024691522628700660907665*sin(q3L)*((7514214926474921*cos(q2L)*((4872700232219253*cos(q1L))/9007199254740992 + (6283307137322267*sin(q1L))/9007199254740992))/36893488147419103232 - sin(q2L)*((6283307137322267*cos(q1L))/9007199254740992 - (4872700232219253*sin(q1L))/9007199254740992)))/42535295865117307932921825928971026432 - (106069577339469832923929692356850887620017617375*cos(q2L)*((4872700232219253*cos(q1L))/9007199254740992 + (6283307137322267*sin(q1L))/9007199254740992))/12554203470773361527671578846415332832204710888928069025792 + (14115856197532180673579726082375*sin(q2L)*((6283307137322267*cos(q1L))/9007199254740992 - (4872700232219253*sin(q1L))/9007199254740992))/340282366920938463463374607431768211456 - (81129635049124235038645691064225*cos(q3L)*((43889380989894851923989405068805*cos(q1L))/81129638414606681695789005144064 + (56594998190739085871744456992395*sin(q1L))/81129638414606681695789005144064))/81129638414606681695789005144064 + (2115063383689692319117831580025*sin(q3L)*((43889380989894851923989405068805*cos(q1L))/81129638414606681695789005144064 + (56594998190739085871744456992395*sin(q1L))/81129638414606681695789005144064))/10384593717069655257060992658440192 - (234819211581865*cos(q3L)*(cos(q2L)*((6283307137322267*cos(q1L))/9007199254740992 - (4872700232219253*sin(q1L))/9007199254740992) + (7514214926474921*sin(q2L)*((4872700232219253*cos(q1L))/9007199254740992 + (6283307137322267*sin(q1L))/9007199254740992))/36893488147419103232))/1152921504606846976 - (67682029681889335677290557259385*cos(q3L)*((7514214926474921*cos(q2L)*((4872700232219253*cos(q1L))/9007199254740992 + (6283307137322267*sin(q1L))/9007199254740992))/36893488147419103232 - sin(q2L)*((6283307137322267*cos(q1L))/9007199254740992 - (4872700232219253*sin(q1L))/9007199254740992)))/332306998946228968225951765070086144))/9007199254740992 + sin(q5L)*(((7514214926474921*cos(q4L))/36893488147419103232 + (4503599440548691*sin(q4L))/4503599627370496)*((7514214926474921*sin(q3L)*((7514214926474921*cos(q2L)*((4872700232219253*cos(q1L))/9007199254740992 + (6283307137322267*sin(q1L))/9007199254740992))/36893488147419103232 - sin(q2L)*((6283307137322267*cos(q1L))/9007199254740992 - (4872700232219253*sin(q1L))/9007199254740992)))/36893488147419103232 + (9007199067919185*sin(q3L)*((43889380989894851923989405068805*cos(q1L))/81129638414606681695789005144064 + (56594998190739085871744456992395*sin(q1L))/81129638414606681695789005144064))/9007199254740992 - cos(q3L)*(cos(q2L)*((6283307137322267*cos(q1L))/9007199254740992 - (4872700232219253*sin(q1L))/9007199254740992) + (7514214926474921*sin(q2L)*((4872700232219253*cos(q1L))/9007199254740992 + (6283307137322267*sin(q1L))/9007199254740992))/36893488147419103232)) - ((9007199067919185*cos(q4L))/9007199254740992 - (234819211581865*sin(q4L))/1152921504606846976)*((329794241748012540206902858004467560228111939405*cos(q1L))/2993155353253689176481146537402947624255349848014848 + (425266980168672787164801917791314326747055225795*sin(q1L))/2993155353253689176481146537402947624255349848014848 - (67682029681889335677290557259385*cos(q2L)*((4872700232219253*cos(q1L))/9007199254740992 + (6283307137322267*sin(q1L))/9007199254740992))/332306998946228968225951765070086144 + (9007199067919185*sin(q2L)*((6283307137322267*cos(q1L))/9007199254740992 - (4872700232219253*sin(q1L))/9007199254740992))/9007199254740992) + (7514214926474921*sin(q4L)*(sin(q3L)*(cos(q2L)*((6283307137322267*cos(q1L))/9007199254740992 - (4872700232219253*sin(q1L))/9007199254740992) + (7514214926474921*sin(q2L)*((4872700232219253*cos(q1L))/9007199254740992 + (6283307137322267*sin(q1L))/9007199254740992))/36893488147419103232) + (9007199067919185*cos(q3L)*((43889380989894851923989405068805*cos(q1L))/81129638414606681695789005144064 + (56594998190739085871744456992395*sin(q1L))/81129638414606681695789005144064))/9007199254740992 + (7514214926474921*cos(q3L)*((7514214926474921*cos(q2L)*((4872700232219253*cos(q1L))/9007199254740992 + (6283307137322267*sin(q1L))/9007199254740992))/36893488147419103232 - sin(q2L)*((6283307137322267*cos(q1L))/9007199254740992 - (4872700232219253*sin(q1L))/9007199254740992)))/36893488147419103232))/36893488147419103232)))/332306998946228968225951765070086144000 + (807520961047489018778067709720399904923771262077295170375712179706208528987338271217011451790113918662491539890779991*cos(q2L)*((4872700232219253*cos(q1L))/9007199254740992 + (6283307137322267*sin(q1L))/9007199254740992))/15760802478557791684911616040057445522031895708186178667179317361698288708598884244565706501953966256322651196122726400000 - (3*cos(q2L)*((6283307137322267*cos(q1L))/9007199254740992 - (4872700232219253*sin(q1L))/9007199254740992))/100 + (27*cos(q6L)*((9007199067919185*sin(q5L)*((516845254133432670685844229576986303733782399690601453662320875*cos(q1L))/113078212145816597093331040047546785012958969400039613319782796882727665664 + (666467732349846997487583938718911583194406904318712922873589125*sin(q1L))/113078212145816597093331040047546785012958969400039613319782796882727665664 - (9007199067919185*sin(q3L)*(cos(q2L)*((6283307137322267*cos(q1L))/9007199254740992 - (4872700232219253*sin(q1L))/9007199254740992) + (7514214926474921*sin(q2L)*((4872700232219253*cos(q1L))/9007199254740992 + (6283307137322267*sin(q1L))/9007199254740992))/36893488147419103232))/9007199254740992 + (1764482024691522628700660907665*sin(q3L)*((7514214926474921*cos(q2L)*((4872700232219253*cos(q1L))/9007199254740992 + (6283307137322267*sin(q1L))/9007199254740992))/36893488147419103232 - sin(q2L)*((6283307137322267*cos(q1L))/9007199254740992 - (4872700232219253*sin(q1L))/9007199254740992)))/42535295865117307932921825928971026432 - (106069577339469832923929692356850887620017617375*cos(q2L)*((4872700232219253*cos(q1L))/9007199254740992 + (6283307137322267*sin(q1L))/9007199254740992))/12554203470773361527671578846415332832204710888928069025792 + (14115856197532180673579726082375*sin(q2L)*((6283307137322267*cos(q1L))/9007199254740992 - (4872700232219253*sin(q1L))/9007199254740992))/340282366920938463463374607431768211456 - (81129635049124235038645691064225*cos(q3L)*((43889380989894851923989405068805*cos(q1L))/81129638414606681695789005144064 + (56594998190739085871744456992395*sin(q1L))/81129638414606681695789005144064))/81129638414606681695789005144064 + (2115063383689692319117831580025*sin(q3L)*((43889380989894851923989405068805*cos(q1L))/81129638414606681695789005144064 + (56594998190739085871744456992395*sin(q1L))/81129638414606681695789005144064))/10384593717069655257060992658440192 - (234819211581865*cos(q3L)*(cos(q2L)*((6283307137322267*cos(q1L))/9007199254740992 - (4872700232219253*sin(q1L))/9007199254740992) + 